simulink model "r_128w_8k_1a_16x_r431"  (R2012b)
settings: Solver=FixedStepDiscrete  SolverMode=SingleTasking  StartTime=0.0  StopTime=5000  RelTol=1e-3
undefined symbols (not defined in the file): Down, pfb_coeff_gen_calc, Up
libraries: xbsIndex_r4 x9410, casper_library_misc x257, casper_library_delays x92, xps_library x57, simulink x16, dspsigops x12, casper_library_flow_control x8, xbsReplacements_r4 x4, casper_library_multipliers x4, casper_library_scopes x2, casper_library_ffts_twiddle x2
(part 1 of 125)
settings Model: ExtModeAutoUpdateStatusClock=off  Creator=Jason Manley  LastModifiedBy=jmanley
settings DataIOCC: SignalLoggingSaveFormat=ModelDataLogs  SaveOutput=off  SaveTime=off
settings OptimizationCC: InitFltsAndDblsToZero=on
settings DebuggingCC: SolverPrmCheckMsg=none  FcnCallInpInsideContextMsg=UseLocalSettings  StrictBusMsg=Warning
settings GRTTargetCC: CombineOutputUpdateFcns=off  GRTInterface=on

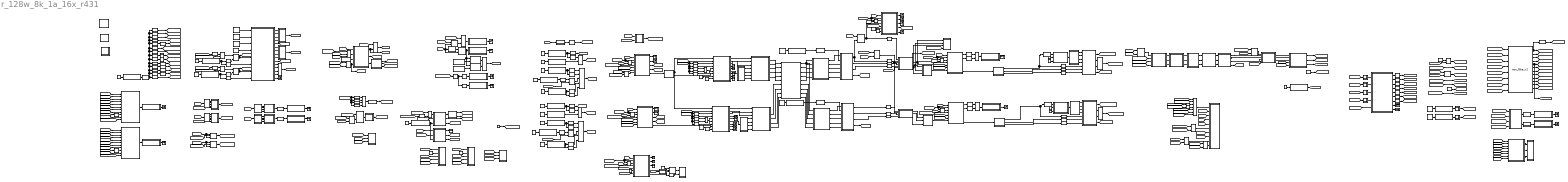
== system r_128w_8k_1a_16x_r431 ==
  note: * A resync command will cause the sync_gen to stop issuing sync pulses.
      | * It will then ignore the next input trigger (1PPS), while sync is flushed through the DSP pipeline.
      | * It will then lock onto the next trigger (1PPS) and issue a sync.
      | * Need a multiple of (pfb_fir taps*LCM(FFT reorder orders) *fft bins/parallel inputs =)
      | (4 * LCM(2,2,2,9) * 2048 / 4) = 9216) for sync_period for simulation
  note: coarse delay logic
  note: Prevent saturation
      | in first stage of FFT
      | by shifting down.
  note: Controls whether there is
      | a shift to the right after
      | multiplication at the
      | respective stage in the
      | fft to prevent
      | overflow.
  note: requantisation
      | to 4 bits
  note: polyphase FIR and FFT
  note: Accept 32 data words from ibob,
      | plus a 1 word header,
      | creating UDP packets of length 33 x 64 bits.
      | This block generates the destination IP address.
  note: Fine delay tracking and
      | fringe stopping
  note: delay tracking and
      | fringe stopping registers
  note: clock and synchronisation
      | info
  note: transient event/RFI debugging infrastructure
  note: data alignment infrastructure to
      | align to within one clock cycle
      | using PPS
  note: input power estimation
      | infrastructure
  note: ADC protection
      | infrastructure
  note: data reordering
  note: packet formation
  note: comms
  note: outputs value to GPIO pin to
      | prove timed register functionality
  note: tvg that can be activated at
      | specific time in data stream
  note: r431 2013-05-17
      | - 8k mode based on r430 1k mode
      | - 4taps
      | - new PFB
      | - new snap blocks
      | - new shared bram
      | - removed snap_xaui and snap_quant to save BRAM
  " System Generator" : xbsIndex_r4/ System Generator  Tag=genX  xilinxfamily=virtex5  part=xc5vsx95t  speed=-1  package=ff1136  synthesis_tool=XST  clock_wrapper=Clock Enables  directory=./r_128w_8k_1a_16x_r431/sysgen  proj_type=Project Navigator  Synth_file=XST Defaults  Impl_file=ISE Defaults  testbench=off  simulink_period=1  sysclk_period=5  dcm_input_clock_period=100  incr_netlist=off  trim_vbits=Everywhere in SubSystem  dbl_ovrd=According to Block Masks  core_generation=According to Block Masks  run_coregen=off  deprecated_control=off  eval_field=0  block_type=sysgen
      settings: block_version=10.1.3
  AddSub : xbsIndex_r4/AddSub  mode=Addition  use_carryin=off  use_carryout=off  en=off  latency=1  precision=User Defined  arith_type=Unsigned  n_bits=15  bin_pt=0  quantization=Truncate  overflow=Saturate  dbl_ovrd=off  use_behavioral_HDL=off  hw_selection=DSP48  pipelined=on  block_type=addsub
  AddSub1 : xbsIndex_r4/AddSub  mode=Addition  use_carryin=off  use_carryout=off  en=off  latency=1  precision=User Defined  arith_type=Unsigned  n_bits=15  bin_pt=0  quantization=Truncate  overflow=Saturate  dbl_ovrd=off  use_behavioral_HDL=off  hw_selection=DSP48  pipelined=on  block_type=addsub
  Concat : xbsIndex_r4/Concat  num_inputs=3  dbl_ovrd=off  block_type=concat
      settings: block_version=10.1.3
  Concat1 : xbsIndex_r4/Concat  num_inputs=5  dbl_ovrd=off  block_type=concat
      settings: block_version=10.1.3
  Concat{2..7,9..10,13..14,21} (11 alike) : xbsIndex_r4/Concat  num_inputs=2  dbl_ovrd=off  block_type=concat
      Concat13 settings: block_version=10.1.3
      Concat14 settings: block_version=10.1.3
      Concat2 settings: block_version=10.1.3
      Concat3 settings: block_version=10.1.3
      Concat7 settings: block_version=10.1.3
      Concat9 settings: block_version=10.1.3
  Concat22 : xbsIndex_r4/Concat  num_inputs=5  dbl_ovrd=off  block_type=concat
      settings: block_version=10.1.3
  Concat8 : xbsIndex_r4/Concat  num_inputs=4  dbl_ovrd=off  block_type=concat
  Constant : Constant  SampleTime=1/4
  Constant1 : xbsIndex_r4/Constant  const=1  gui_display_data_type=Fixed-point  arith_type=Boolean  n_bits=1  bin_pt=0  preci_type=Single  exp_width=8  frac_width=24  explicit_period=off  period=1  equ=P=C  opselect=C  inp2=PCIN>>17  opr=+  inp1=P  carry=CIN  dbl_ovrd=off  block_type=constant
      settings: block_version=11.4
  Constant10 : xbsIndex_r4/Constant  const=0  gui_display_data_type=Fixed-point  arith_type=Unsigned  n_bits=64  bin_pt=0  preci_type=Single  exp_width=8  frac_width=24  explicit_period=off  period=1  equ=P=C  opselect=C  inp2=PCIN>>17  opr=+  inp1=P  carry=CIN  dbl_ovrd=off  block_type=constant
      settings: block_version=11.4
  Constant11 : xbsIndex_r4/Constant  const=0  gui_display_data_type=Fixed-point  arith_type=Boolean  n_bits=64  bin_pt=0  preci_type=Single  exp_width=8  frac_width=24  explicit_period=off  period=1  equ=P=C  opselect=C  inp2=PCIN>>17  opr=+  inp1=P  carry=CIN  dbl_ovrd=off  block_type=constant
      settings: block_version=11.4
  Constant{4,8,12,15..16,32} (6 alike) : Constant  Value=8
  Constant{3,9,13,18,27,33,40,48} (8 alike) : Constant  Value=0
  Constant{14,19..20,22,35} (5 alike) : xbsIndex_r4/Constant  const=0  gui_display_data_type=Fixed-point  arith_type=Boolean  n_bits=1  bin_pt=0  preci_type=Single  exp_width=8  frac_width=24  explicit_period=on  period=1  equ=P=C  opselect=C  inp2=PCIN>>17  opr=+  inp1=P  carry=CIN  dbl_ovrd=off  block_type=constant
      Constant14 settings: block_version=11.4
      Constant19 settings: block_version=11.4
      Constant20 settings: block_version=11.3
      Constant22 settings: block_version=11.4
      Constant35 settings: block_version=11.4
  Constant17 : xbsIndex_r4/Constant  const=0  gui_display_data_type=Fixed-point  arith_type=Unsigned  n_bits=1  bin_pt=0  preci_type=Single  exp_width=8  frac_width=24  explicit_period=on  period=1  equ=P=C  opselect=C  inp2=PCIN>>17  opr=+  inp1=P  carry=CIN  dbl_ovrd=off  block_type=constant
      settings: block_version=11.4
  Constant2 : xbsIndex_r4/Constant  const=12*2*8192*2^14  gui_display_data_type=Fixed-point  arith_type=Unsigned  n_bits=32  bin_pt=0  preci_type=Single  exp_width=8  frac_width=24  explicit_period=off  period=1  equ=P=C  opselect=C  inp2=PCIN>>17  opr=+  inp1=P  carry=CIN  dbl_ovrd=off  block_type=constant
  Constant21 : xbsIndex_r4/Constant  const=0  gui_display_data_type=Fixed-point  arith_type=Unsigned  n_bits=1  bin_pt=0  preci_type=Single  exp_width=8  frac_width=24  explicit_period=on  period=1  equ=P=C  opselect=C  inp2=PCIN>>17  opr=+  inp1=P  carry=CIN  dbl_ovrd=off  block_type=constant
      settings: block_version=11.4
  Constant23 : xbsIndex_r4/Constant  const=0  gui_display_data_type=Boolean  arith_type=Boolean  n_bits=1  bin_pt=0  preci_type=Single  exp_width=8  frac_width=24  explicit_period=off  period=1  equ=P=C  opselect=C  inp2=PCIN>>17  opr=+  inp1=P  carry=CIN  dbl_ovrd=off  block_type=constant
      settings: block_version=11.4
  Constant24 : xbsIndex_r4/Constant  const=1  gui_display_data_type=Fixed-point  arith_type=Boolean  n_bits=1  bin_pt=0  preci_type=Single  exp_width=8  frac_width=24  explicit_period=off  period=1  equ=P=C  opselect=C  inp2=PCIN>>17  opr=+  inp1=P  carry=CIN  dbl_ovrd=off  block_type=constant
      settings: block_version=11.4
  Constant25 : Constant  Value=100
  Constant29 : Constant  Value=20
  Constant34 : xbsIndex_r4/Constant  const=0  gui_display_data_type=Fixed-point  arith_type=Boolean  n_bits=16  bin_pt=14  preci_type=Single  exp_width=8  frac_width=24  explicit_period=on  period=1  equ=P=C  opselect=C  inp2=PCIN>>17  opr=+  inp1=P  carry=CIN  dbl_ovrd=off  block_type=constant
      settings: block_version=11.4
  Constant36 : xbsIndex_r4/Constant  const=800000000/4+1  gui_display_data_type=Fixed-point  arith_type=Unsigned  n_bits=32  bin_pt=0  preci_type=Single  exp_width=8  frac_width=24  explicit_period=on  period=1  equ=P=C  opselect=C  inp2=PCIN>>17  opr=+  inp1=P  carry=CIN  dbl_ovrd=off  block_type=constant
      settings: block_version=11.4
  Constant37 : xbsIndex_r4/Constant  const=800000000/4-1  gui_display_data_type=Fixed-point  arith_type=Unsigned  n_bits=32  bin_pt=0  preci_type=Single  exp_width=8  frac_width=24  explicit_period=on  period=1  equ=P=C  opselect=C  inp2=PCIN>>17  opr=+  inp1=P  carry=CIN  dbl_ovrd=off  block_type=constant
      settings: block_version=11.4
  Constant38 : xbsIndex_r4/Constant  const=1  gui_display_data_type=Fixed-point  arith_type=Unsigned  n_bits=1  bin_pt=0  preci_type=Single  exp_width=8  frac_width=24  explicit_period=on  period=1  equ=P=C  opselect=C  inp2=PCIN>>17  opr=+  inp1=P  carry=CIN  dbl_ovrd=off  block_type=constant
      settings: block_version=11.4
  Constant41 : xbsIndex_r4/Constant  const=0  gui_display_data_type=Fixed-point  arith_type=Unsigned  n_bits=64  bin_pt=0  preci_type=Single  exp_width=8  frac_width=24  explicit_period=off  period=1  equ=P=C  opselect=C  inp2=PCIN>>17  opr=+  inp1=P  carry=CIN  dbl_ovrd=off  block_type=constant
      settings: block_version=11.4
  Constant46 : xbsIndex_r4/Constant  const=0  gui_display_data_type=Fixed-point  arith_type=Boolean  n_bits=64  bin_pt=0  preci_type=Single  exp_width=8  frac_width=24  explicit_period=off  period=1  equ=P=C  opselect=C  inp2=PCIN>>17  opr=+  inp1=P  carry=CIN  dbl_ovrd=off  block_type=constant
      settings: block_version=11.4
  Constant5 : xbsIndex_r4/Constant  const=1  gui_display_data_type=Fixed-point  arith_type=Boolean  n_bits=1  bin_pt=0  preci_type=Single  exp_width=8  frac_width=24  explicit_period=on  period=1  equ=P=C  opselect=C  inp2=PCIN>>17  opr=+  inp1=P  carry=CIN  dbl_ovrd=off  block_type=constant
  Constant6 : Constant  Value=20
  Constant7 : xbsIndex_r4/Constant  const=0  gui_display_data_type=Fixed-point  arith_type=Boolean  n_bits=16  bin_pt=14  preci_type=Single  exp_width=8  frac_width=24  explicit_period=on  period=1  equ=P=C  opselect=C  inp2=PCIN>>17  opr=+  inp1=P  carry=CIN  dbl_ovrd=off  block_type=constant
      settings: block_version=11.4
  Convert{4..7} (4 alike) : xbsIndex_r4/Convert  gui_display_data_type=Fixed-point  arith_type=Unsigned  n_bits=16  bin_pt=0  float_type=Single  exp_bits=8  fraction_bits=24  quantization=Truncate  overflow=Wrap  en=off  latency=0  dbl_ovrd=off  pipeline=on  block_type=convert
      settings: block_version=11.4
  Counter1 : xbsIndex_r4/Counter  cnt_type=Free Running  cnt_to=Inf  operation=Up  start_count=1  cnt_by_val=1  arith_type=Unsigned  n_bits=32  bin_pt=0  load_pin=off  rst=on  en=off  explicit_period=on  period=1  dbl_ovrd=off  use_behavioral_HDL=off  implementation=Fabric  use_rpm=on  block_type=counter
  Counter2 : xbsIndex_r4/Counter  cnt_type=Free Running  cnt_to=Inf  operation=Up  start_count=0  cnt_by_val=1  arith_type=Unsigned  n_bits=12  bin_pt=0  load_pin=off  rst=on  en=off  explicit_period=on  period=1  dbl_ovrd=off  use_behavioral_HDL=off  implementation=Fabric  block_type=counter
      settings: block_version=11.4
  Counter3 : xbsIndex_r4/Counter  cnt_type=Free Running  cnt_to=Inf  operation=Up  start_count=0  cnt_by_val=1  arith_type=Unsigned  n_bits=31  bin_pt=0  load_pin=off  rst=on  en=on  explicit_period=on  period=1  dbl_ovrd=off  use_behavioral_HDL=off  implementation=DSP48  use_rpm=on  block_type=counter
  Counter8 : xbsIndex_r4/Counter  cnt_type=Free Running  cnt_to=Inf  operation=Up  start_count=0  cnt_by_val=1  arith_type=Unsigned  n_bits=12  bin_pt=0  load_pin=off  rst=on  en=off  explicit_period=on  period=1  dbl_ovrd=off  use_behavioral_HDL=off  implementation=Fabric  block_type=counter
      settings: block_version=11.4
  Delay : xbsIndex_r4/Delay  rst=off  infoeditControl=Selection of Reset will increase slice count due to use of real FFs and instead of SRLs  en=off  latency=1  dbl_ovrd=off  reg_retiming=off  block_type=delay
      settings: block_version=11.4
  Delay1 : Subsystem  AncestorBlock=casper_library/Delays/pipeline  mask(pipeline){latency=1}
      mask help:
      | An explicitly laid-out delay line to avoid mapping to SRL16s
      | for use in pipelining to help achieve timing closure.
      mask init:
      | pipeline_init(gcb, 'latency', latency);
      mask Display:
      | port_label('input', 1, 'd');
      | port_label('output', 1, 'q');
      | disp(['Z^-', num2str(latency)]);
  Delay10 : Subsystem  AncestorBlock=casper_library/Delays/pipeline  mask(pipeline){latency=1}
      mask help:
      | An explicitly laid-out delay line to avoid mapping to SRL16s
      | for use in pipelining to help achieve timing closure.
      mask init:
      | pipeline_init(gcb, 'latency', latency);
      mask Display:
      | port_label('input', 1, 'd');
      | port_label('output', 1, 'q');
      | disp(['Z^-', num2str(latency)]);
  Delay100 : Subsystem  AncestorBlock=casper_library/Delays/pipeline  mask(pipeline){latency=2}
      mask help:
      | An explicitly laid-out delay line to avoid mapping to SRL16s
      | for use in pipelining to help achieve timing closure.
      mask init:
      | pipeline_init(gcb, 'latency', latency);
      mask Display:
      | port_label('input', 1, 'd');
      | port_label('output', 1, 'q');
      | disp(['Z^-', num2str(latency)]);
  Delay11 : Subsystem  AncestorBlock=casper_library/Delays/pipeline  mask(pipeline){latency=1}
      mask help:
      | An explicitly laid-out delay line to avoid mapping to SRL16s
      | for use in pipelining to help achieve timing closure.
      mask init:
      | pipeline_init(gcb, 'latency', latency);
      mask Display:
      | port_label('input', 1, 'd');
      | port_label('output', 1, 'q');
      | disp(['Z^-', num2str(latency)]);
  Delay12 : xbsIndex_r4/Delay  rst=off  infoeditControl=Selection of Reset will increase slice count due to use of real FFs and instead of SRLs  en=off  latency=1  dbl_ovrd=off  reg_retiming=off  block_type=delay
      settings: block_version=11.4
  Delay{13,15..19} (6 alike) : xbsIndex_r4/Delay  rst=off  infoeditControl=Selection of Reset will increase slice count due to use of real FFs and instead of SRLs  en=off  latency=3  dbl_ovrd=off  reg_retiming=off  block_type=delay
      settings: block_version=11.4
  Delay14 : Subsystem  AncestorBlock=casper_library/Delays/pipeline  mask(pipeline){latency=2}
      mask help:
      | An explicitly laid-out delay line to avoid mapping to SRL16s
      | for use in pipelining to help achieve timing closure.
      mask init:
      | pipeline_init(gcb, 'latency', latency);
      mask Display:
      | port_label('input', 1, 'd');
      | port_label('output', 1, 'q');
      | disp(['Z^-', num2str(latency)]);
  Delay2 : Subsystem  AncestorBlock=casper_library/Delays/pipeline  mask(pipeline){latency=2}
      mask help:
      | An explicitly laid-out delay line to avoid mapping to SRL16s
      | for use in pipelining to help achieve timing closure.
      mask init:
      | pipeline_init(gcb, 'latency', latency);
      mask Display:
      | port_label('input', 1, 'd');
      | port_label('output', 1, 'q');
      | disp(['Z^-', num2str(latency)]);
  Delay{20..22,24..27} (7 alike) : xbsIndex_r4/Delay  rst=off  infoeditControl=Selection of Reset will increase slice count due to use of real FFs and instead of SRLs  en=off  latency=4  dbl_ovrd=off  reg_retiming=off  block_type=delay
      settings: block_version=11.4
  Delay23 : Subsystem  AncestorBlock=casper_library/Delays/pipeline  mask(pipeline){latency=1}
      mask help:
      | An explicitly laid-out delay line to avoid mapping to SRL16s
      | for use in pipelining to help achieve timing closure.
      mask init:
      | pipeline_init(gcb, 'latency', latency);
      mask Display:
      | port_label('input', 1, 'd');
      | port_label('output', 1, 'q');
      | disp(['Z^-', num2str(latency)]);
  Delay28 : xbsIndex_r4/Delay  rst=off  infoeditControl=Selection of Reset will increase slice count due to use of real FFs and instead of SRLs  en=off  latency=1  dbl_ovrd=off  reg_retiming=on  block_type=delay
  Delay3 : Subsystem  AncestorBlock=casper_library/Delays/pipeline  mask(pipeline){latency=1}
      mask help:
      | An explicitly laid-out delay line to avoid mapping to SRL16s
      | for use in pipelining to help achieve timing closure.
      mask init:
      | pipeline_init(gcb, 'latency', latency);
      mask Display:
      | port_label('input', 1, 'd');
      | port_label('output', 1, 'q');
      | disp(['Z^-', num2str(latency)]);
  Delay31 : Subsystem  AncestorBlock=casper_library/Delays/pipeline  mask(pipeline){latency=1}
      mask help:
      | An explicitly laid-out delay line to avoid mapping to SRL16s
      | for use in pipelining to help achieve timing closure.
      mask init:
      | pipeline_init(gcb, 'latency', latency);
      mask Display:
      | port_label('input', 1, 'd');
      | port_label('output', 1, 'q');
      | disp(['Z^-', num2str(latency)]);
  Delay33 : Subsystem  AncestorBlock=casper_library/Delays/pipeline  mask(pipeline){latency=1}
      mask help:
      | An explicitly laid-out delay line to avoid mapping to SRL16s
      | for use in pipelining to help achieve timing closure.
      mask init:
      | pipeline_init(gcb, 'latency', latency);
      mask Display:
      | port_label('input', 1, 'd');
      | port_label('output', 1, 'q');
      | disp(['Z^-', num2str(latency)]);
  Delay34 : Subsystem  AncestorBlock=casper_library/Delays/pipeline  mask(pipeline){latency=1}
      mask help:
      | An explicitly laid-out delay line to avoid mapping to SRL16s
      | for use in pipelining to help achieve timing closure.
      mask init:
      | pipeline_init(gcb, 'latency', latency);
      mask Display:
      | port_label('input', 1, 'd');
      | port_label('output', 1, 'q');
      | disp(['Z^-', num2str(latency)]);
  Delay4 : Subsystem  AncestorBlock=casper_library/Delays/pipeline  mask(pipeline){latency=1}
      mask help:
      | An explicitly laid-out delay line to avoid mapping to SRL16s
      | for use in pipelining to help achieve timing closure.
      mask init:
      | pipeline_init(gcb, 'latency', latency);
      mask Display:
      | port_label('input', 1, 'd');
      | port_label('output', 1, 'q');
      | disp(['Z^-', num2str(latency)]);
  Delay5 : Subsystem  AncestorBlock=casper_library/Delays/pipeline  mask(pipeline){latency=1}
      mask help:
      | An explicitly laid-out delay line to avoid mapping to SRL16s
      | for use in pipelining to help achieve timing closure.
      mask init:
      | pipeline_init(gcb, 'latency', latency);
      mask Display:
      | port_label('input', 1, 'd');
      | port_label('output', 1, 'q');
      | disp(['Z^-', num2str(latency)]);
  Delay6 : xbsIndex_r4/Delay  rst=off  infoeditControl=Selection of Reset will increase slice count due to use of real FFs and instead of SRLs  en=off  latency=1  dbl_ovrd=off  reg_retiming=on  block_type=delay
  Delay64 : Subsystem  AncestorBlock=casper_library/Delays/pipeline  mask(pipeline){latency=2}
      mask help:
      | An explicitly laid-out delay line to avoid mapping to SRL16s
      | for use in pipelining to help achieve timing closure.
      mask init:
      | pipeline_init(gcb, 'latency', latency);
      mask Display:
      | port_label('input', 1, 'd');
      | port_label('output', 1, 'q');
      | disp(['Z^-', num2str(latency)]);
  Delay7 : xbsIndex_r4/Delay  rst=off  infoeditControl=Selection of Reset will increase slice count due to use of real FFs and instead of SRLs  en=off  latency=1  dbl_ovrd=off  reg_retiming=on  block_type=delay
  Delay71 : Subsystem  AncestorBlock=casper_library/Delays/pipeline  mask(pipeline){latency=2}
      mask help:
      | An explicitly laid-out delay line to avoid mapping to SRL16s
      | for use in pipelining to help achieve timing closure.
      mask init:
      | pipeline_init(gcb, 'latency', latency);
      mask Display:
      | port_label('input', 1, 'd');
      | port_label('output', 1, 'q');
      | disp(['Z^-', num2str(latency)]);
  Delay72 : Subsystem  AncestorBlock=casper_library/Delays/pipeline  mask(pipeline){latency=2}
      mask help:
      | An explicitly laid-out delay line to avoid mapping to SRL16s
      | for use in pipelining to help achieve timing closure.
      mask init:
      | pipeline_init(gcb, 'latency', latency);
      mask Display:
      | port_label('input', 1, 'd');
      | port_label('output', 1, 'q');
      | disp(['Z^-', num2str(latency)]);
  Delay8 : xbsIndex_r4/Delay  rst=off  infoeditControl=Selection of Reset will increase slice count due to use of real FFs and instead of SRLs  en=off  latency=1  dbl_ovrd=off  reg_retiming=off  block_type=delay
      settings: block_version=11.4
  Delay9 : Subsystem  AncestorBlock=casper_library/Delays/pipeline  mask(pipeline){latency=1}
      mask help:
      | An explicitly laid-out delay line to avoid mapping to SRL16s
      | for use in pipelining to help achieve timing closure.
      mask init:
      | pipeline_init(gcb, 'latency', latency);
      mask Display:
      | port_label('input', 1, 'd');
      | port_label('output', 1, 'q');
      | disp(['Z^-', num2str(latency)]);
  Inverter{,1..6} (7 alike) : xbsIndex_r4/Inverter  en=off  latency=0  dbl_ovrd=off  block_type=inv
      settings: block_version=11.4
  Logical : xbsIndex_r4/Logical  logical_function=OR  inputs=4  en=off  latency=0  precision=Full  arith_type=Unsigned  n_bits=16  bin_pt=0  align_bp=on  dbl_ovrd=off  block_type=logical
  Logical1 : xbsIndex_r4/Logical  logical_function=AND  inputs=2  en=off  latency=0  precision=Full  arith_type=Unsigned  n_bits=8  bin_pt=2  align_bp=on  dbl_ovrd=off  block_type=logical
      settings: xl_area=[0, 0, 0, 0, 0, 0, 0]
  Logical10 : xbsIndex_r4/Logical  logical_function=AND  inputs=2  en=off  latency=0  precision=Full  arith_type=Unsigned  n_bits=16  bin_pt=0  align_bp=on  dbl_ovrd=off  block_type=logical
  Logical{3..4,6,9,11..15,19..21} (12 alike) : xbsIndex_r4/Logical  logical_function=OR  inputs=2  en=off  latency=0  precision=Full  arith_type=Unsigned  n_bits=16  bin_pt=0  align_bp=on  dbl_ovrd=off  block_type=logical
      Logical11 settings: block_version=11.4
      Logical12 settings: block_version=11.4
      Logical13 settings: block_version=11.4
      Logical15 settings: block_version=11.4
      Logical19 settings: block_version=11.4
      Logical20 settings: block_version=11.4
      Logical21 settings: block_version=11.4
  Logical16 : xbsIndex_r4/Logical  logical_function=OR  inputs=2  en=off  latency=1  precision=Full  arith_type=Unsigned  n_bits=16  bin_pt=0  align_bp=on  dbl_ovrd=off  block_type=logical
  Logical17 : xbsIndex_r4/Logical  logical_function=OR  inputs=2  en=off  latency=1  precision=Full  arith_type=Unsigned  n_bits=16  bin_pt=0  align_bp=on  dbl_ovrd=off  block_type=logical
  Logical2 : xbsIndex_r4/Logical  logical_function=OR  inputs=2  en=off  latency=1  precision=Full  arith_type=Unsigned  n_bits=8  bin_pt=2  align_bp=on  dbl_ovrd=off  block_type=logical
      settings: xl_area=[0, 0, 0, 0, 0, 0, 0]
  Logical5 : xbsIndex_r4/Logical  logical_function=AND  inputs=2  en=off  latency=0  precision=Full  arith_type=Unsigned  n_bits=16  bin_pt=0  align_bp=on  dbl_ovrd=off  block_type=logical
  Logical7 : xbsIndex_r4/Logical  logical_function=OR  inputs=7  en=off  latency=1  precision=Full  arith_type=Unsigned  n_bits=16  bin_pt=0  align_bp=on  dbl_ovrd=off  block_type=logical
  Logical8 : xbsIndex_r4/Logical  logical_function=AND  inputs=2  en=off  latency=0  precision=Full  arith_type=Unsigned  n_bits=16  bin_pt=0  align_bp=on  dbl_ovrd=off  block_type=logical
  Pulse Generator : DiscretePulseGenerator  Amplitude=0.75  Period=2^11  PhaseDelay=11  SampleTime=1/4
  Pulse Generator1 : DiscretePulseGenerator  Period=2^8  PhaseDelay=9+13+2^8  SampleTime=1/4
  Pulse Generator2 : DiscretePulseGenerator  Amplitude=0.5  Period=2^11  PhaseDelay=9+14+2^8  SampleTime=1/4
  Recombine channels : Subsystem  mask{channel_bits=8}
      mask prompts: channel_bits "Bits per channel:"
      mask help: FFT data per polarisation is in the form of two channels of n-bit data concatenated together. This block splits given inputs of this form and groups outputs by channel, not polarisation.
  Register{,1..3,19} (5 alike) : xbsIndex_r4/Register  init=0  rst=off  en=on  dbl_ovrd=off  block_type=register
      Register settings: block_version=11.4
      Register1 settings: block_version=11.4
      Register2 settings: block_version=11.4
      Register3 settings: block_version=11.4
  Register4 : xbsIndex_r4/Register  init=0  rst=on  en=on  dbl_ovrd=off  block_type=register
      settings: block_version=11.4
  Register5 : xbsIndex_r4/Register  init=0  rst=on  en=on  dbl_ovrd=off  block_type=register
  Register9 : xbsIndex_r4/Register  init=0  rst=on  en=on  dbl_ovrd=off  block_type=register
  Relational : xbsIndex_r4/Relational  mode=a>b  en=off  latency=1  dbl_ovrd=off  block_type=relational
  Relational1 : xbsIndex_r4/Relational  mode=a<b  en=off  latency=1  dbl_ovrd=off  block_type=relational
  Slice : xbsIndex_r4/Slice  nbits=32  boolean_output=off  mode=Lower Bit Location + Width  bit1=0  base1=MSB of Input  bit0=0  base0=LSB of Input  dbl_ovrd=off  block_type=slice
  Slice1 : xbsIndex_r4/Slice  nbits=32  boolean_output=off  mode=Lower Bit Location + Width  bit1=0  base1=MSB of Input  bit0=32  base0=LSB of Input  dbl_ovrd=off  block_type=slice
  Slice{2,4,13,28,37,73} (6 alike) : xbsIndex_r4/Slice  nbits=16  boolean_output=off  mode=Lower Bit Location + Width  bit1=0  base1=MSB of Input  bit0=0  base0=LSB of Input  dbl_ovrd=off  block_type=slice
      settings: infoedit="Extracts a given range of bits from each input sample and presents it at the output.  The output type is ordinarily unsigned with binary point at zero, but can be Boolean when the slice is one bit wide.<P><P>Hardware notes: In hardware this block costs nothing."  block_version=10.1.3
  Slice14 : xbsIndex_r4/Slice  nbits=32  boolean_output=off  mode=Lower Bit Location + Width  bit1=0  base1=MSB of Input  bit0=0  base0=LSB of Input  dbl_ovrd=off  block_type=slice
  Slice15 : xbsIndex_r4/Slice  nbits=16  boolean_output=off  mode=Lower Bit Location + Width  bit1=0  base1=MSB of Input  bit0=0*16  base0=LSB of Input  dbl_ovrd=off  block_type=slice
      settings: block_version=10.1.3
  Slice16 : xbsIndex_r4/Slice  nbits=16  boolean_output=off  mode=Lower Bit Location + Width  bit1=0  base1=MSB of Input  bit0=16*3+15  base0=LSB of Input  dbl_ovrd=off  block_type=slice
      settings: block_version=10.1.3
  Slice17 : xbsIndex_r4/Slice  nbits=16  boolean_output=off  mode=Lower Bit Location + Width  bit1=0  base1=MSB of Input  bit0=16*1  base0=LSB of Input  dbl_ovrd=off  block_type=slice
      settings: block_version=10.1.3
  Slice18 : xbsIndex_r4/Slice  nbits=15  boolean_output=off  mode=Lower Bit Location + Width  bit1=0  base1=MSB of Input  bit0=16*2  base0=LSB of Input  dbl_ovrd=off  block_type=slice
      settings: block_version=10.1.3
  Slice19 : xbsIndex_r4/Slice  nbits=16  boolean_output=off  mode=Lower Bit Location + Width  bit1=0  base1=MSB of Input  bit0=16*2+15  base0=LSB of Input  dbl_ovrd=off  block_type=slice
      settings: block_version=10.1.3
  Slice20 : xbsIndex_r4/Slice  nbits=16  boolean_output=off  mode=Lower Bit Location + Width  bit1=0  base1=MSB of Input  bit0=0*16  base0=LSB of Input  dbl_ovrd=off  block_type=slice
      settings: block_version=10.1.3
  Slice21 : xbsIndex_r4/Slice  nbits=16  boolean_output=off  mode=Lower Bit Location + Width  bit1=0  base1=MSB of Input  bit0=16*3+15  base0=LSB of Input  dbl_ovrd=off  block_type=slice
      settings: block_version=10.1.3
  Slice22 : xbsIndex_r4/Slice  nbits=16  boolean_output=off  mode=Lower Bit Location + Width  bit1=0  base1=MSB of Input  bit0=16*1  base0=LSB of Input  dbl_ovrd=off  block_type=slice
      settings: block_version=10.1.3
  Slice23 : xbsIndex_r4/Slice  nbits=15  boolean_output=off  mode=Lower Bit Location + Width  bit1=0  base1=MSB of Input  bit0=16*2  base0=LSB of Input  dbl_ovrd=off  block_type=slice
      settings: block_version=10.1.3
  Slice24 : xbsIndex_r4/Slice  nbits=16  boolean_output=off  mode=Lower Bit Location + Width  bit1=0  base1=MSB of Input  bit0=16*2+15  base0=LSB of Input  dbl_ovrd=off  block_type=slice
      settings: block_version=10.1.3
  Slice{3,5,25,31} (4 alike) : xbsIndex_r4/Slice  nbits=16  boolean_output=off  mode=Lower Bit Location + Width  bit1=0  base1=MSB of Input  bit0=16  base0=LSB of Input  dbl_ovrd=off  block_type=slice
      Slice25 settings: infoedit="Extracts a given range of bits from each input sample and presents it at the output.  The output type is ordinarily unsigned with binary point at zero, but can be Boolean when the slice is one bit wide.<P><P>Hardware notes: In hardware this block costs nothing."  block_version=10.1.3
      Slice3 settings: infoedit="Extracts a given range of bits from each input sample and presents it at the output.  The output type is ordinarily unsigned with binary point at zero, but can be Boolean when the slice is one bit wide.<P><P>Hardware notes: In hardware this block costs nothing."  block_version=10.1.3
      Slice31 settings: block_version=10.1.3
      Slice5 settings: block_version=10.1.3
  Slice{6,26..27,38} (4 alike) : xbsIndex_r4/Slice  nbits=15  boolean_output=off  mode=Lower Bit Location + Width  bit1=0  base1=MSB of Input  bit0=0  base0=LSB of Input  dbl_ovrd=off  block_type=slice
      settings: block_version=10.1.3
  Slice{7,29,32..33} (4 alike) : xbsIndex_r4/Slice  nbits=1  boolean_output=on  mode=Upper Bit Location + Width  bit1=0  base1=MSB of Input  bit0=0  base0=LSB of Input  dbl_ovrd=off  block_type=slice
      Slice32 settings: block_version=10.1.3
      Slice7 settings: block_version=10.1.3
  Slice30 : xbsIndex_r4/Slice  nbits=6  boolean_output=off  mode=Lower Bit Location + Width  bit1=0  base1=MSB of Input  bit0=0  base0=LSB of Input  dbl_ovrd=off  block_type=slice
  Slice34 : xbsIndex_r4/Slice  nbits=6  boolean_output=off  mode=Lower Bit Location + Width  bit1=0  base1=MSB of Input  bit0=0  base0=LSB of Input  dbl_ovrd=off  block_type=slice
  Slice35 : xbsIndex_r4/Slice  nbits=1  boolean_output=on  mode=Lower Bit Location + Width  bit1=0  base1=MSB of Input  bit0=3  base0=LSB of Input  dbl_ovrd=off  block_type=slice
  Slice36 : xbsIndex_r4/Slice  nbits=1  boolean_output=on  mode=Lower Bit Location + Width  bit1=0  base1=MSB of Input  bit0=2  base0=LSB of Input  dbl_ovrd=off  block_type=slice
  Slice40 : xbsIndex_r4/Slice  nbits=1  boolean_output=on  mode=Lower Bit Location + Width  bit1=0  base1=MSB of Input  bit0=1  base0=LSB of Input  dbl_ovrd=off  block_type=slice
  Slice45 : xbsIndex_r4/Slice  nbits=1  boolean_output=on  mode=Lower Bit Location + Width  bit1=0  base1=MSB of Input  bit0=0  base0=LSB of Input  dbl_ovrd=off  block_type=slice
  Slice78 : xbsIndex_r4/Slice  nbits=1  boolean_output=on  mode=Lower Bit Location + Width  bit1=0  base1=MSB of Input  bit0=0  base0=LSB of Input  dbl_ovrd=off  block_type=slice
      settings: block_version=10.1.3
  Split channels : Subsystem  mask{channel_bits=8}
      mask prompts: channel_bits "Bits per channel:"
      mask help: FFT data per polarisation is in the form of two channels of n-bit data concatenated together. This block splits given inputs of this form and groups outputs by channel, not polarisation.
  Subsystem1 : Subsystem
  Subsystem3 : Subsystem
  Subsystem4 : Subsystem
  Subsystem5 : Subsystem
  Subsystem7 : Subsystem
  Terminator{,1..19,21,23,25..29,35..44} (37 alike) : Terminator
  X-engine reorder : Subsystem  mask{num_channels_bits=13, num_xengines_bits=4, num_data_bits=16, bram_latency=0}
      mask prompts: num_channels_bits "Number of channels (2^?)"; num_xengines_bits "Number of X-engines (2^?)"; num_data_bits "Incoming data width in bits (per channel, 2 pols):"; bram_latency "BRAM latency"
      mask help:
      | Interleaves the parallel output (even and odd channels) of an FFT between multiple X-engines in a correlator.
      | i.e. X0 will get F0, F1, F2... and Xn will get F(nChan/nXeng), F(nChan/nXeng) + 1, etc.
  XSG core config : xps_library/XSG core config  Tag=xps:xsg  hw_sys=ROACH:sx95t  clk_src=adc0_clk  ROACH_clk_src=adc0_clk  ROACH2_clk_src=adc0_clk  clk_rate=800/4  sample_period=1  synthesis_tool=XST
  a0_fd0 : xps_library/software register  Tag=xps:sw_reg  io_dir=From Processor  arith_type=Unsigned  bitwidth=32  bin_pt=0  sample_period=1  gw_name=r_128w_8k_1a_16x_r431_a0_fd0_user_data_out
      link override r_128w_8k_1a_16x_r430_a0_fd0_user_data_out: arith_type=Unsigned  n_bits=32  bin_pt=0  period=1
      link override r_128w_8k_1a_16x_r431_a0_fd0_user_data_out: arith_type=Unsigned  n_bits=32  bin_pt=0  period=1
  a0_fd1 : xps_library/software register  Tag=xps:sw_reg  io_dir=From Processor  arith_type=Unsigned  bitwidth=32  bin_pt=0  sample_period=1  gw_name=r_128w_8k_1a_16x_r431_a0_fd1_user_data_out
      link override r_128w_8k_1a_16x_r430_a0_fd1_user_data_out: arith_type=Unsigned  n_bits=32  bin_pt=0  period=1
      link override r_128w_8k_1a_16x_r431_a0_fd1_user_data_out: arith_type=Unsigned  n_bits=32  bin_pt=0  period=1
  a0p0_1st_shift : Subsystem  mask{shift=1, latency=0}
      mask prompts: shift "Number bits to shift right by"; latency "Shift latency"
  a0p1_1st_shift : Subsystem  mask{shift=1, latency=0}
      mask prompts: shift "Number bits to shift right by"; latency "Shift latency"
  a1_fd0 : xps_library/software register  Tag=xps:sw_reg  io_dir=From Processor  arith_type=Unsigned  bitwidth=32  bin_pt=0  sample_period=1  gw_name=r_128w_8k_1a_16x_r431_a1_fd0_user_data_out
      link override r_128w_8k_1a_16x_r430_a1_fd0_user_data_out: arith_type=Unsigned  n_bits=32  bin_pt=0  period=1
      link override r_128w_8k_1a_16x_r431_a1_fd0_user_data_out: arith_type=Unsigned  n_bits=32  bin_pt=0  period=1
  a1_fd1 : xps_library/software register  Tag=xps:sw_reg  io_dir=From Processor  arith_type=Unsigned  bitwidth=32  bin_pt=0  sample_period=1  gw_name=r_128w_8k_1a_16x_r431_a1_fd1_user_data_out
      link override r_128w_8k_1a_16x_r430_a1_fd1_user_data_out: arith_type=Unsigned  n_bits=32  bin_pt=0  period=1
      link override r_128w_8k_1a_16x_r431_a1_fd1_user_data_out: arith_type=Unsigned  n_bits=32  bin_pt=0  period=1
  adc_ctrl0 : xps_library/software register  Tag=xps:sw_reg  io_dir=From Processor  arith_type=Unsigned  bitwidth=32  bin_pt=0  sample_period=1  gw_name=r_128w_8k_1a_16x_r431_adc_ctrl0_user_data_out
      link override r_128w_8k_1a_16x_r430_adc_ctrl0_user_data_out: arith_type=Unsigned  n_bits=32  bin_pt=0  period=1
      link override r_128w_8k_1a_16x_r431_adc_ctrl0_user_data_out: arith_type=Unsigned  n_bits=32  bin_pt=0  period=1
  adc_ctrl1 : xps_library/software register  Tag=xps:sw_reg  io_dir=From Processor  arith_type=Unsigned  bitwidth=32  bin_pt=0  sample_period=1  gw_name=r_128w_8k_1a_16x_r431_adc_ctrl1_user_data_out
      link override r_128w_8k_1a_16x_r430_adc_ctrl1_user_data_out: arith_type=Unsigned  n_bits=32  bin_pt=0  period=1
      link override r_128w_8k_1a_16x_r431_adc_ctrl1_user_data_out: arith_type=Unsigned  n_bits=32  bin_pt=0  period=1
  adc_scope : Subsystem
  adc_snap0 : Subsystem  Tag=casper:snapshot  AncestorBlock=casper_library_scopes/snapshot  mask(snapshot){storage=bram, dram_dimm=1, dram_clock=200, nsamples=11, data_width=32, offset=on, circap=on, value=on, use_dsp48=off}
      mask prompts: storage "Storage medium"; dram_dimm "DRAM dimm"; dram_clock "DRAM clock rate"; nsamples "Number of Samples (2^?)"; data_width "Data width"; offset "Start delay support"; circap "Circular capture support"; value "Extra value capture support"; use_dsp48 "Use DSP48s to implement counters"
      mask help:
      | Standard snap block, but with the following optional extras;
      |  1) Optionally delay the fabric trigger by a user-specified number of valids.
      |  2) Capture continuously after a trigger until a stop pulse is received. Data is captured into BRAM continuously, with old data being overwritten until a stop command is received. Then stop capturing when memory is filled. This enables you to get some data before and some data after the stop pulse. Use the 'tr_en_cnt' register to determine where you are in your vector. 'Addr' register's MSb now indicates 'busy capturing'.
      |  3) Optionally capture a value on an input port to a register at the same time as the first data sample.
      |  4) Implement counters using DSP48Es to save resources.
      mask init:
      | snapshot_init(gcb, ...
      |     'storage', storage, ...
      |     'dram_dimm', dram_dimm, ...
      |     'dram_clock', dram_clock, ...
      |     'nsamples', nsamples, ...
      |     'data_width', data_width, ...
      |     'offset', offset, ...
      |     'circap', circap, ...
      |     'value', value, ...
      |     'use_dsp48', use_dsp48);
      mask TypeOptions storage: bram | dram
      mask Callback storage: snapshot_callback();
      mask TypeOptions dram_dimm: 1 | 2 | 3 | 4
      mask TypeOptions dram_clock: 200 | 250 | 266 | 300 | 333
      mask TypeOptions data_width: 8 | 16 | 32 | 64 | 128
  adc_snap1 : Subsystem  Tag=casper:snapshot  AncestorBlock=casper_library_scopes/snapshot  mask(snapshot){storage=bram, dram_dimm=1, dram_clock=200, nsamples=11, data_width=32, offset=on, circap=on, value=on, use_dsp48=off}
      mask prompts: storage "Storage medium"; dram_dimm "DRAM dimm"; dram_clock "DRAM clock rate"; nsamples "Number of Samples (2^?)"; data_width "Data width"; offset "Start delay support"; circap "Circular capture support"; value "Extra value capture support"; use_dsp48 "Use DSP48s to implement counters"
      mask help:
      | Standard snap block, but with the following optional extras;
      |  1) Optionally delay the fabric trigger by a user-specified number of valids.
      |  2) Capture continuously after a trigger until a stop pulse is received. Data is captured into BRAM continuously, with old data being overwritten until a stop command is received. Then stop capturing when memory is filled. This enables you to get some data before and some data after the stop pulse. Use the 'tr_en_cnt' register to determine where you are in your vector. 'Addr' register's MSb now indicates 'busy capturing'.
      |  3) Optionally capture a value on an input port to a register at the same time as the first data sample.
      |  4) Implement counters using DSP48Es to save resources.
      mask init: same as r_128w_8k_1a_16x_r431/adc_snap0
      mask TypeOptions storage: bram | dram
      mask Callback storage: snapshot_callback();
      mask TypeOptions dram_dimm: 1 | 2 | 3 | 4
      mask TypeOptions dram_clock: 200 | 250 | 266 | 300 | 333
      mask TypeOptions data_width: 8 | 16 | 32 | 64 | 128
  adc_sum_sq0 : Subsystem  Tag=xps:sw_reg  mask{io_dir=To Processor, arith_type=Unsigned, bitwidth=32, bin_pt=0, sample_period=1, latency=0}
      mask prompts: io_dir "I/O direction"; arith_type "Data Type"; bitwidth "Data bitwidth"; bin_pt "Data binary point"; sample_period "Sample period"
      mask init:
      | gw_name = clear_name(gcb);
      | config.source = str2func('software_register_init');
      | config.toplevel = gcb;
      | xBlock( config, {io_dir, arith_type, bitwidth, bin_pt, ... 
      |     sample_period, gw_name, latency});
      mask TypeOptions io_dir: From Processor | To Processor
      mask TypeOptions arith_type: Unsigned | Signed  (2's comp)
  adc_sum_sq1 : Subsystem  Tag=xps:sw_reg  mask{io_dir=To Processor, arith_type=Unsigned, bitwidth=32, bin_pt=0, sample_period=1, latency=0}
      mask prompts: io_dir "I/O direction"; arith_type "Data Type"; bitwidth "Data bitwidth"; bin_pt "Data binary point"; sample_period "Sample period"
      mask init:
      | gw_name = clear_name(gcb);
      | config.source = str2func('software_register_init');
      | config.toplevel = gcb;
      | xBlock( config, {io_dir, arith_type, bitwidth, bin_pt, ... 
      |     sample_period, gw_name, latency});
      mask TypeOptions io_dir: From Processor | To Processor
      mask TypeOptions arith_type: Unsigned | Signed  (2's comp)
  arm1 : xbsIndex_r4/Slice  nbits=1  boolean_output=on  mode=Lower Bit Location + Width  bit1=0  base1=MSB of Input  bit0=2  base0=LSB of Input  dbl_ovrd=off  block_type=slice
      settings: block_version=10.1.3
  arm10 : xbsIndex_r4/Slice  nbits=1  boolean_output=on  mode=Lower Bit Location + Width  bit1=0  base1=MSB of Input  bit0=12  base0=LSB of Input  dbl_ovrd=off  block_type=slice
      settings: block_version=10.1.3
  arm11 : xbsIndex_r4/Slice  nbits=1  boolean_output=on  mode=Lower Bit Location + Width  bit1=0  base1=MSB of Input  bit0=13  base0=LSB of Input  dbl_ovrd=off  block_type=slice
      settings: block_version=10.1.3
  arm12 : xbsIndex_r4/Slice  nbits=1  boolean_output=on  mode=Lower Bit Location + Width  bit1=0  base1=MSB of Input  bit0=4  base0=LSB of Input  dbl_ovrd=off  block_type=slice
      settings: block_version=10.1.3
  arm2 : xbsIndex_r4/Slice  nbits=1  boolean_output=on  mode=Lower Bit Location + Width  bit1=0  base1=MSB of Input  bit0=3  base0=LSB of Input  dbl_ovrd=off  block_type=slice
      settings: block_version=10.1.3
  arm3 : xbsIndex_r4/Slice  nbits=1  boolean_output=on  mode=Lower Bit Location + Width  bit1=0  base1=MSB of Input  bit0=16  base0=LSB of Input  dbl_ovrd=off  block_type=slice
      settings: block_version=10.1.3
  arm4 : xbsIndex_r4/Slice  nbits=1  boolean_output=on  mode=Lower Bit Location + Width  bit1=0  base1=MSB of Input  bit0=17  base0=LSB of Input  dbl_ovrd=off  block_type=slice
      settings: block_version=10.1.3
  arm5 : xbsIndex_r4/Slice  nbits=1  boolean_output=on  mode=Lower Bit Location + Width  bit1=0  base1=MSB of Input  bit0=18  base0=LSB of Input  dbl_ovrd=off  block_type=slice
      settings: block_version=10.1.3
  arm6 : xbsIndex_r4/Slice  nbits=1  boolean_output=on  mode=Lower Bit Location + Width  bit1=0  base1=MSB of Input  bit0=19  base0=LSB of Input  dbl_ovrd=off  block_type=slice
      settings: block_version=10.1.3
  arm7 : xbsIndex_r4/Slice  nbits=1  boolean_output=on  mode=Lower Bit Location + Width  bit1=0  base1=MSB of Input  bit0=20  base0=LSB of Input  dbl_ovrd=off  block_type=slice
      settings: block_version=10.1.3
  arm8 : xbsIndex_r4/Slice  nbits=1  boolean_output=on  mode=Lower Bit Location + Width  bit1=0  base1=MSB of Input  bit0=9  base0=LSB of Input  dbl_ovrd=off  block_type=slice
      settings: block_version=10.1.3
  arm9 : xbsIndex_r4/Slice  nbits=1  boolean_output=on  mode=Lower Bit Location + Width  bit1=0  base1=MSB of Input  bit0=8  base0=LSB of Input  dbl_ovrd=off  block_type=slice
      settings: block_version=10.1.3
  auto_shutoff0 : Subsystem  mask{bits_in=8, bin_pt_in=7, clk_freq=200, acc_time=20, max_power=1/sqrt(2)}
      mask prompts: bits_in "Input bits"; bin_pt_in "Input binary point"; clk_freq "Clock frequency (MHz)"; acc_time "Window (ms)"; max_power "Max power allowed"
  auto_shutoff1 : Subsystem  mask{bits_in=8, bin_pt_in=7, clk_freq=200, acc_time=20, max_power=1/sqrt(2)}
      mask prompts: bits_in "Input bits"; bin_pt_in "Input binary point"; clk_freq "Clock frequency (MHz)"; acc_time "Window (ms)"; max_power "Max power allowed"
  board_id : xps_library/software register  Tag=xps:sw_reg  io_dir=From Processor  arith_type=Unsigned  bitwidth=32  bin_pt=0  sample_period=1  gw_name=r_128w_8k_1a_16x_r431_board_id_user_data_out
      link override r_128w_8k_1a_16x_r430_board_id_user_data_out: arith_type=Unsigned  n_bits=32  bin_pt=0  period=1
      link override r_128w_8k_1a_16x_r431_board_id_user_data_out: arith_type=Unsigned  n_bits=32  bin_pt=0  period=1
  bus_create : Subsystem  AncestorBlock=casper_library_flow_control/bus_create  mask(bus_create){inputNum=3}
      mask prompts: inputNum "Number of inputs:"
      mask init:
      | bus_create_init(gcb,...
      |     'inputNum', inputNum);
  bus_create1 : Subsystem  AncestorBlock=casper_library_flow_control/bus_create  mask(bus_create){inputNum=3}
      mask prompts: inputNum "Number of inputs:"
      mask init:
      | bus_create_init(gcb,...
      |     'inputNum', inputNum);
  bus_expand : Subsystem  AncestorBlock=casper_library_flow_control/bus_expand  mask(bus_expand){mode=divisions of arbitrary size, outputNum=2, outputWidth=[1                                     32], outputBinaryPt=[0                                      0], outputArithmeticType=[2                                      0], outputToWorkspace=off, variablePrefix=out, outputToModelAsWell=on}
      mask prompts: outputNum "Number of outputs:"; outputWidth "Output width [msb ... lsb]:"; outputBinaryPt "Output binary point position [msb ... lsb]:"; outputArithmeticType "Output arithmetic type (ufix=0, fix=1, bool=2) [msb ... lsb]:"; outputToWorkspace "Output to workspace?"; variablePrefix "Variable name prefix:"; outputToModelAsWell "Output to model as well?"
      mask help:
      | Expands a 'bus' made using a bus_create or Xilinx
      | concat block.
      | The input will be divided into the specified number
      | of outputs with the specified arithmetic types.
      | Divisions are made from most significant bit.
      mask init:
      | bus_expand_init(gcb,...
      |     'mode', mode, ...
      |     'outputNum', outputNum, ...
      |     'outputWidth', outputWidth, ...
      |     'outputBinaryPt', outputBinaryPt, ...
      |     'outputArithmeticType', outputArithmeticType, ...
      |     'outputToWorkspace', outputToWorkspace, ...
      |     'variablePrefix', variablePrefix, ...
      |     'outputToModelAsWell', outputToModelAsWell);
      settings: AttributesFormatString=2 outputs
      mask TypeOptions mode: divisions of equal size | divisions of arbitrary size
      mask Callback mode: bus_expand_callback();
      mask Callback outputWidth: bus_expand_callback();
      mask Callback outputToWorkspace: bus_expand_callback();
  bus_expand1 : Subsystem  AncestorBlock=casper_library_flow_control/bus_expand  mask(bus_expand){mode=divisions of arbitrary size, outputNum=3, outputWidth=[1                                     36                                     36], outputBinaryPt=[0                                      0                                      0], outputArithmeticType=[2                                      0                                      0], outputToWorkspace=off, variablePrefix=out, outputToModelAsWell=on}
      mask prompts: outputNum "Number of outputs:"; outputWidth "Output width [msb ... lsb]:"; outputBinaryPt "Output binary point position [msb ... lsb]:"; outputArithmeticType "Output arithmetic type (ufix=0, fix=1, bool=2) [msb ... lsb]:"; outputToWorkspace "Output to workspace?"; variablePrefix "Variable name prefix:"; outputToModelAsWell "Output to model as well?"
      mask help:
      | Expands a 'bus' made using a bus_create or Xilinx
      | concat block.
      | The input will be divided into the specified number
      | of outputs with the specified arithmetic types.
      | Divisions are made from most significant bit.
      mask init: same as r_128w_8k_1a_16x_r431/bus_expand
      settings: AttributesFormatString=3 outputs
      mask TypeOptions mode: divisions of equal size | divisions of arbitrary size
      mask Callback mode: bus_expand_callback();
      mask Callback outputWidth: bus_expand_callback();
      mask Callback outputToWorkspace: bus_expand_callback();
  bus_expand2 : Subsystem  AncestorBlock=casper_library_flow_control/bus_expand  mask(bus_expand){mode=divisions of equal size, outputNum=4, outputWidth=16, outputBinaryPt=1, outputArithmeticType=1, outputToWorkspace=off, variablePrefix=out, outputToModelAsWell=on}
      mask prompts: outputNum "Number of outputs:"; outputWidth "Output width:"; outputBinaryPt "Output binary point position:"; outputArithmeticType "Output arithmetic type (ufix=0, fix=1, bool=2):"; outputToWorkspace "Output to workspace?"; variablePrefix "Variable name prefix:"; outputToModelAsWell "Output to model as well?"
      mask help:
      | Expands a 'bus' made using a bus_create or Xilinx
      | concat block.
      | The input will be divided into the specified number
      | of outputs with the specified arithmetic types.
      | Divisions are made from most significant bit.
      mask init: same as r_128w_8k_1a_16x_r431/bus_expand
      settings: AttributesFormatString=4 outputs
      mask TypeOptions mode: divisions of equal size | divisions of arbitrary size
      mask Callback mode: bus_expand_callback();
      mask Callback outputWidth: bus_expand_callback();
      mask Callback outputToWorkspace: bus_expand_callback();
  bus_expand3 : Subsystem  AncestorBlock=casper_library_flow_control/bus_expand  mask(bus_expand){mode=divisions of arbitrary size, outputNum=3, outputWidth=[1                                     36                                     36], outputBinaryPt=[0                                      0                                      0], outputArithmeticType=[2                                      0                                      0], outputToWorkspace=off, variablePrefix=out, outputToModelAsWell=on}
      mask prompts: outputNum "Number of outputs:"; outputWidth "Output width [msb ... lsb]:"; outputBinaryPt "Output binary point position [msb ... lsb]:"; outputArithmeticType "Output arithmetic type (ufix=0, fix=1, bool=2) [msb ... lsb]:"; outputToWorkspace "Output to workspace?"; variablePrefix "Variable name prefix:"; outputToModelAsWell "Output to model as well?"
      mask help:
      | Expands a 'bus' made using a bus_create or Xilinx
      | concat block.
      | The input will be divided into the specified number
      | of outputs with the specified arithmetic types.
      | Divisions are made from most significant bit.
      mask init: same as r_128w_8k_1a_16x_r431/bus_expand
      settings: AttributesFormatString=3 outputs
      mask TypeOptions mode: divisions of equal size | divisions of arbitrary size
      mask Callback mode: bus_expand_callback();
      mask Callback outputWidth: bus_expand_callback();
      mask Callback outputToWorkspace: bus_expand_callback();
  bus_expand4 : Subsystem  AncestorBlock=casper_library_flow_control/bus_expand  mask(bus_expand){mode=divisions of equal size, outputNum=4, outputWidth=16, outputBinaryPt=1, outputArithmeticType=1, outputToWorkspace=off, variablePrefix=out, outputToModelAsWell=on}
      mask prompts: outputNum "Number of outputs:"; outputWidth "Output width:"; outputBinaryPt "Output binary point position:"; outputArithmeticType "Output arithmetic type (ufix=0, fix=1, bool=2):"; outputToWorkspace "Output to workspace?"; variablePrefix "Variable name prefix:"; outputToModelAsWell "Output to model as well?"
      mask help:
      | Expands a 'bus' made using a bus_create or Xilinx
      | concat block.
      | The input will be divided into the specified number
      | of outputs with the specified arithmetic types.
      | Divisions are made from most significant bit.
      mask init: same as r_128w_8k_1a_16x_r431/bus_expand
      settings: AttributesFormatString=4 outputs
      mask TypeOptions mode: divisions of equal size | divisions of arbitrary size
      mask Callback mode: bus_expand_callback();
      mask Callback outputWidth: bus_expand_callback();
      mask Callback outputToWorkspace: bus_expand_callback();
  bus_expand5 : Subsystem  AncestorBlock=casper_library_flow_control/bus_expand  mask(bus_expand){mode=divisions of arbitrary size, outputNum=2, outputWidth=[1                                     32], outputBinaryPt=[0                                      0], outputArithmeticType=[2                                      0], outputToWorkspace=off, variablePrefix=out, outputToModelAsWell=on}
      mask prompts: outputNum "Number of outputs:"; outputWidth "Output width [msb ... lsb]:"; outputBinaryPt "Output binary point position [msb ... lsb]:"; outputArithmeticType "Output arithmetic type (ufix=0, fix=1, bool=2) [msb ... lsb]:"; outputToWorkspace "Output to workspace?"; variablePrefix "Variable name prefix:"; outputToModelAsWell "Output to model as well?"
      mask help:
      | Expands a 'bus' made using a bus_create or Xilinx
      | concat block.
      | The input will be divided into the specified number
      | of outputs with the specified arithmetic types.
      | Divisions are made from most significant bit.
      mask init: same as r_128w_8k_1a_16x_r431/bus_expand
      settings: AttributesFormatString=2 outputs
      mask TypeOptions mode: divisions of equal size | divisions of arbitrary size
      mask Callback mode: bus_expand_callback();
      mask Callback outputWidth: bus_expand_callback();
      mask Callback outputToWorkspace: bus_expand_callback();
  bus_expand6 : Subsystem  AncestorBlock=casper_library_flow_control/bus_expand  mask(bus_expand){mode=divisions of arbitrary size, outputNum=3, outputWidth=[1                                     32                                     32], outputBinaryPt=[0                                      0                                      0], outputArithmeticType=[2                                      0                                      0], outputToWorkspace=off, variablePrefix=out, outputToModelAsWell=on}
      mask prompts: outputNum "Number of outputs:"; outputWidth "Output width [msb ... lsb]:"; outputBinaryPt "Output binary point position [msb ... lsb]:"; outputArithmeticType "Output arithmetic type (ufix=0, fix=1, bool=2) [msb ... lsb]:"; outputToWorkspace "Output to workspace?"; variablePrefix "Variable name prefix:"; outputToModelAsWell "Output to model as well?"
      mask help:
      | Expands a 'bus' made using a bus_create or Xilinx
      | concat block.
      | The input will be divided into the specified number
      | of outputs with the specified arithmetic types.
      | Divisions are made from most significant bit.
      mask init: same as r_128w_8k_1a_16x_r431/bus_expand
      settings: AttributesFormatString=3 outputs
      mask TypeOptions mode: divisions of equal size | divisions of arbitrary size
      mask Callback mode: bus_expand_callback();
      mask Callback outputWidth: bus_expand_callback();
      mask Callback outputToWorkspace: bus_expand_callback();
  calc_adc_sum_sq : Subsystem
  calc_adc_sum_sq1 : Subsystem
  cd_local_time : Subsystem
  cd_tr0 : Subsystem  mask{cnt_bits=8, time_bits=48}
      mask prompts: cnt_bits "Bits in status counters"; time_bits "No LSBs in time to compare"
  cd_tr1 : Subsystem  mask{cnt_bits=8, time_bits=48}
      mask prompts: cnt_bits "Bits in status counters"; time_bits "No LSBs in time to compare"
  clk_frequency : Subsystem  Tag=xps:sw_reg  mask{io_dir=To Processor, arith_type=Unsigned, bitwidth=32, bin_pt=0, sample_period=1, latency=0}
      link override convert: arith_type=Unsigned  n_bits=32  bin_pt=0
      mask prompts: io_dir "I/O direction"; arith_type "Data Type"; bitwidth "Data bitwidth"; bin_pt "Data binary point"; sample_period "Sample period"
      mask init:
      | gw_name = clear_name(gcb);
      | config.source = str2func('software_register_init');
      | config.toplevel = gcb;
      | xBlock( config, {io_dir, arith_type, bitwidth, bin_pt, ... 
      |     sample_period, gw_name, latency});
      mask TypeOptions io_dir: From Processor | To Processor
      mask TypeOptions arith_type: Unsigned | Signed  (2's comp)
  coarse_delay0 : xps_library/software register  Tag=xps:sw_reg  io_dir=From Processor  arith_type=Unsigned  bitwidth=32  bin_pt=0  sample_period=1  gw_name=r_128w_8k_1a_16x_r431_coarse_delay0_user_data_out
      link override r_128w_8k_1a_16x_r430_coarse_delay0_user_data_out: arith_type=Unsigned  n_bits=32  bin_pt=0  period=1
      link override r_128w_8k_1a_16x_r431_coarse_delay0_user_data_out: arith_type=Unsigned  n_bits=32  bin_pt=0  period=1
  coarse_delay1 : xps_library/software register  Tag=xps:sw_reg  io_dir=From Processor  arith_type=Unsigned  bitwidth=32  bin_pt=0  sample_period=1  gw_name=r_128w_8k_1a_16x_r431_coarse_delay1_user_data_out
      link override r_128w_8k_1a_16x_r430_coarse_delay1_user_data_out: arith_type=Unsigned  n_bits=32  bin_pt=0  period=1
      link override r_128w_8k_1a_16x_r431_coarse_delay1_user_data_out: arith_type=Unsigned  n_bits=32  bin_pt=0  period=1
  control : xps_library/software register  Tag=xps:sw_reg  io_dir=From Processor  arith_type=Unsigned  bitwidth=32  bin_pt=0  sample_period=1  gw_name=r_128w_8k_1a_16x_r431_control_user_data_out
      link override r_128w_8k_1a_16x_r430_control_user_data_out: arith_type=Unsigned  n_bits=32  bin_pt=0  period=1
      link override r_128w_8k_1a_16x_r431_control_user_data_out: arith_type=Unsigned  n_bits=32  bin_pt=0  period=1
  convert : Subsystem
  ct : Subsystem  mask{input_bits=13, output_bits=7, parallel_bits=1, which_qdr=qdr0}
      mask prompts: input_bits "Input vector length (total 2^?):"; output_bits "Output packet size (2^? samples):"; parallel_bits "Parallel Input channels per polarisation (2^?)"; which_qdr "QDR to use:"
      mask init:
      | set_param([gcb, '/qdr_ct'], 'which_qdr', which_qdr);
      mask TypeOptions which_qdr: qdr0 | qdr1
  ct_tvg : Subsystem  mask{num_channels_bits=13, channel_bits=8}
      mask prompts: num_channels_bits "Number of channels (2^?):"; channel_bits "Bits per channel:"
  decat0 : Subsystem
  decat1 : Subsystem
  decat2 : Subsystem
  decat3 : Subsystem
  delay_gen0 : Subsystem  mask{fft_len=10, phase_bits=16, max_fringe_rate=23, min_fringe_rate=38, delay_bits=16+15, delay_bin_pt=16, max_delay_rate=23, min_delay_rate=38, add_latency=1, lookup_bits=11, cd_bits=15}
      mask prompts: fft_len "FFT size (2^?)"; phase_bits "Input phase resolution (2*pi/2^? radians)"; max_fringe_rate "Max fringe update rate (1/2^? radians/sample)"; min_fringe_rate "Min (non-zero) fringe rate (1/2^? radians/sample)"; delay_bits "Input delay resolution (bits)"; delay_bin_pt "Input delay binary point"; max_delay_rate "Max delay update rate (1/2^? samples/sample)"; min_delay_rate "Min (non-zero) delay update rate (1/2^? samples/sample)"; add_latency "Add latency"; lookup_bits "DDS lookup table resolution (2*pi/2^?)"; cd_bits "Coarse delay range (2^? bits)"
  delay_gen1 : Subsystem  mask{fft_len=10, phase_bits=16, max_fringe_rate=23, min_fringe_rate=38, delay_bits=16+15, delay_bin_pt=16, max_delay_rate=23, min_delay_rate=38, add_latency=1, lookup_bits=11, cd_bits=15}
      mask prompts: fft_len "FFT size (2^?)"; phase_bits "Input phase resolution (2*pi/2^? radians)"; max_fringe_rate "Max fringe update rate (1/2^? radians/sample)"; min_fringe_rate "Min (non-zero) fringe rate (1/2^? radians/sample)"; delay_bits "Input delay resolution (bits)"; delay_bin_pt "Input delay binary point"; max_delay_rate "Max delay update rate (1/2^? samples/sample)"; min_delay_rate "Min (non-zero) delay update rate (1/2^? samples/sample)"; add_latency "Add latency"; lookup_bits "DDS lookup table resolution (2*pi/2^?)"; cd_bits "Coarse delay range (2^? bits)"
  delay_tr_status0 : Subsystem  Tag=xps:sw_reg  mask{io_dir=To Processor, arith_type=Unsigned, bitwidth=32, bin_pt=0, sample_period=1, latency=0}
      link override convert: arith_type=Unsigned  n_bits=32  bin_pt=0
      mask prompts: io_dir "I/O direction"; arith_type "Data Type"; bitwidth "Data bitwidth"; bin_pt "Data binary point"; sample_period "Sample period"
      mask init:
      | gw_name = clear_name(gcb);
      | config.source = str2func('software_register_init');
      | config.toplevel = gcb;
      | xBlock( config, {io_dir, arith_type, bitwidth, bin_pt, ... 
      |     sample_period, gw_name, latency});
      mask TypeOptions io_dir: From Processor | To Processor
      mask TypeOptions arith_type: Unsigned | Signed  (2's comp)
  delay_tr_status1 : Subsystem  Tag=xps:sw_reg  mask{io_dir=To Processor, arith_type=Unsigned, bitwidth=32, bin_pt=0, sample_period=1, latency=0}
      link override convert: arith_type=Unsigned  n_bits=32  bin_pt=0
      mask prompts: io_dir "I/O direction"; arith_type "Data Type"; bitwidth "Data bitwidth"; bin_pt "Data binary point"; sample_period "Sample period"
      mask init:
      | gw_name = clear_name(gcb);
      | config.source = str2func('software_register_init');
      | config.toplevel = gcb;
      | xBlock( config, {io_dir, arith_type, bitwidth, bin_pt, ... 
      |     sample_period, gw_name, latency});
      mask TypeOptions io_dir: From Processor | To Processor
      mask TypeOptions arith_type: Unsigned | Signed  (2's comp)
  delay_wideband_prog0 : Subsystem  AncestorBlock=casper_library/Delays/delay_wideband_prog  mask(delay_wideband_prog){max_delay=32768, n_inputs_bits=2, bram_latency=2, bram_type=Dual Port}
      mask prompts: max_delay "Max Delay (Sample Clks)"; n_inputs_bits "Number of Simultaneous Inputs(2^?)"; bram_latency "BRAM Latency"; bram_type "Select type of BRAM"
      mask init:
      | delay_wideband_prog_init(gcb,...
      |     'max_delay',max_delay,...
      |     'n_inputs_bits',n_inputs_bits,...
      |     'bram_latency',bram_latency,...
      |     'bram_type',bram_type);
      mask TypeOptions bram_type: Single Port | Dual Port
  delay_wideband_prog1 : Subsystem  AncestorBlock=casper_library/Delays/delay_wideband_prog  mask(delay_wideband_prog){max_delay=32768, n_inputs_bits=2, bram_latency=2, bram_type=Dual Port}
      mask prompts: max_delay "Max Delay (Sample Clks)"; n_inputs_bits "Number of Simultaneous Inputs(2^?)"; bram_latency "BRAM Latency"; bram_type "Select type of BRAM"
      mask init:
      | delay_wideband_prog_init(gcb,...
      |     'max_delay',max_delay,...
      |     'n_inputs_bits',n_inputs_bits,...
      |     'bram_latency',bram_latency,...
      |     'bram_type',bram_type);
      mask TypeOptions bram_type: Single Port | Dual Port
  edge_detect : Subsystem  AncestorBlock=casper_library_misc/edge_detect  mask(edge_detect){edge=Falling, polarity=Active High, x_in=[0 0.08 0.08 0.16 0.16 0.24 0.24 0.32 0.32 0.4], y_in=[1  1 -1 -1 -1 -1 -1 -1 -1 -1], x_out=[0.6 0.68 0.68 0.76 0.76 0.84 0.84 0.92 0.92 1], y_out=[-1 -1  1  1 -1 -1 -1 -1 -1 -1]}
      mask prompts: edge "Edge Type"; polarity "Output Polarity"; x_in "Input X Positions"; y_in "Input Y Positions"; x_out "Output X Positions"; y_out "Output Y Positions"
      mask help: Output is active for one-cycle after each edge of the specified type (i.e. rising, falling or both).
      mask init:
      | edge_detect_init(gcb,...
      |     'edge',edge,...
      |     'polarity',polarity,...
      |     'x_in',x_in,...
      |     'x_out',x_out,...
      |     'y_in',y_in,...
      |     'y_out',y_out);
      | 
      | x_in_num=str2num(getfield(getfield(get_param(gcb,'UserData'),'parameters'),'x_in'));
      | x_out_num=str2num(getfield(getfield(get_param(gcb,'UserData'),'parameters'),'x_out'));
      | y_in_num=str2num(getfield(getfield(get_param(gcb,'UserData'),'parameters'),'y_in'));
      | y_out_num=str2num(getfield(getfield(get_param(gcb,'UserData'),'parameters'),'y_out'));
      settings: AttributesFormatString=|
      | falling edges
      | active high
      mask Help: Output is active for one-cycle after each edge of the specified type (i.e. rising, falling, or both).  Latency is zero.
      mask TypeOptions edge: Rising | Falling | Both
      mask TypeOptions polarity: Active High | Active Low
      mask Display:
      | plot(x_in_num,0.5+y_in_num*0.2);
      | plot(x_out_num,0.5+y_out_num*0.2);
  edge_detect1 : casper_library_misc/edge_detect  edge=Rising  polarity=Active High  x_in=[0 0.08 0.08 0.16 0.16 0.24 0.24 0.32 0.32 0.4]  y_in="[-1 -1  1  1  1  1  1  1  1  1]"  x_out=[0.6 0.68 0.68 0.76 0.76 0.84 0.84 0.92 0.92 1]  y_out="[-1 -1  1  1 -1 -1 -1 -1 -1 -1]"
  edge_detect2 : Subsystem  AncestorBlock=casper_library_misc/edge_detect  mask(edge_detect){edge=Rising, polarity=Active High, x_in=[0 0.08 0.08 0.16 0.16 0.24 0.24 0.32 0.32 0.4], y_in=[-1 -1  1  1  1  1  1  1  1  1], x_out=[0.6 0.68 0.68 0.76 0.76 0.84 0.84 0.92 0.92 1], y_out=[-1 -1  1  1 -1 -1 -1 -1 -1 -1]}
      mask prompts: edge "Edge Type"; polarity "Output Polarity"; x_in "Input X Positions"; y_in "Input Y Positions"; x_out "Output X Positions"; y_out "Output Y Positions"
      mask help: Output is active for one-cycle after each edge of the specified type (i.e. rising, falling or both).
      mask init: same as r_128w_8k_1a_16x_r431/edge_detect
      settings: AttributesFormatString=|
      | rising edges
      | active high
      mask Help: Output is active for one-cycle after each edge of the specified type (i.e. rising, falling, or both).  Latency is zero.
      mask TypeOptions edge: Rising | Falling | Both
      mask TypeOptions polarity: Active High | Active Low
      mask Display:
      | plot(x_in_num,0.5+y_in_num*0.2);
      | plot(x_out_num,0.5+y_out_num*0.2);
  eq0 : Subsystem  Tag=xps:bram  AncestorBlock=xps_library/Shared BRAM  mask{arith_type=Unsigned, addr_width=12, data_width=64, reg_prim_output=on, reg_core_output=on, optimization=Minimum_Area, data_bin_pt=0, init_vals=[0:2^10-1], sample_rate=1}
      mask prompts: arith_type "Output Data Type"; addr_width "Address width"; data_width "Data Width"; reg_prim_output "Register Primitive Output"; reg_core_output "Register Core Output"; data_bin_pt "Data Binary Point"; init_vals "Initial 32-bit values (simulation only)"; sample_rate "Sample rate"
      mask init:
      | shared_bram_mask;
      mask TypeOptions arith_type: Unsigned | Signed  (2's comp)
      mask TypeOptions data_width: 8 | 16 | 32 | 64 | 128
      mask TypeOptions optimization: Minimum_Area | Low_Power
  eq1 : Subsystem  Tag=xps:bram  AncestorBlock=xps_library/Shared BRAM  mask{arith_type=Unsigned, addr_width=12, data_width=64, reg_prim_output=on, reg_core_output=on, optimization=Minimum_Area, data_bin_pt=0, init_vals=[0:2^10-1], sample_rate=1}
      mask prompts: arith_type "Output Data Type"; addr_width "Address width"; data_width "Data Width"; reg_prim_output "Register Primitive Output"; reg_core_output "Register Core Output"; data_bin_pt "Data Binary Point"; init_vals "Initial 32-bit values (simulation only)"; sample_rate "Sample rate"
      mask init:
      | shared_bram_mask;
      mask TypeOptions arith_type: Unsigned | Signed  (2's comp)
      mask TypeOptions data_width: 8 | 16 | 32 | 64 | 128
      mask TypeOptions optimization: Minimum_Area | Low_Power
  err_clear_sim3 : Constant  Value=0
  err_clear_sim4 : Constant  Value=0
  fd_fs_tvg0 : Subsystem  mask{bit_width=18, bin_pt=17, constant=1/16}
      mask prompts: bit_width "bit width"; bin_pt "binary point"
  fd_fs_tvg1 : Subsystem  mask{bit_width=18, bin_pt=17, val=1/16}
      mask prompts: bit_width "bit width"; bin_pt "binary point"; val "constant"
  fd_local_time : Subsystem
  fd_tr0 : Subsystem  mask{cnt_bits=8, time_bits=48}
      mask prompts: cnt_bits "Bits in status counters"; time_bits "No LSBs in time to compare"
  fd_tr1 : Subsystem  mask{cnt_bits=8, time_bits=48}
      mask prompts: cnt_bits "Bits in status counters"; time_bits "No LSBs in time to compare"
  fft_shift0 : xps_library/software register  Tag=xps:sw_reg  io_dir=From Processor  arith_type=Unsigned  bitwidth=32  bin_pt=0  sample_period=1  gw_name=r_128w_8k_1a_16x_r431_fft_shift0_user_data_out
      link override r_128w_8k_1a_16x_r430_fft_shift0_user_data_out: arith_type=Unsigned  n_bits=32  bin_pt=0  period=1
      link override r_128w_8k_1a_16x_r431_fft_shift0_user_data_out: arith_type=Unsigned  n_bits=32  bin_pt=0  period=1
  fft_shift1 : xps_library/software register  Tag=xps:sw_reg  io_dir=From Processor  arith_type=Unsigned  bitwidth=32  bin_pt=0  sample_period=1  gw_name=r_128w_8k_1a_16x_r431_fft_shift1_user_data_out
      link override r_128w_8k_1a_16x_r430_fft_shift1_user_data_out: arith_type=Unsigned  n_bits=32  bin_pt=0  period=1
      link override r_128w_8k_1a_16x_r431_fft_shift1_user_data_out: arith_type=Unsigned  n_bits=32  bin_pt=0  period=1
  fft_wideband_real0 : Subsystem  AncestorBlock=casper_library_ffts/fft_wideband_real  mask(fft_wideband_real){FFTSize=14, n_inputs=2, input_bit_width=18, coeff_bit_width=18, unscramble=on, add_latency=2, mult_latency=2, bram_latency=2, conv_latency=2, input_latency=0, biplex_direct_latency=0, quantization=Round  (unbiased: Even Values), overflow=Wrap, arch=Virtex5, opt_target=logic, coeffs_bit_limit=10, delays_bit_limit=10, mult_spec=1, hardcode_shifts=off, shift_schedule=, dsp48_adders=on}
      mask prompts: FFTSize "Size of FFT: (2^? pts)"; n_inputs "Number of Simultaneous Inputs: (2^?)"; input_bit_width "Input/Output Bit Width"; coeff_bit_width "Coefficient Bit Width"; unscramble "Unscramble output (ie, put channels in canonical order)"; add_latency "Add Latency"; mult_latency "Mult Latency"; bram_latency "BRAM Latency"; conv_latency "Convert Latency"; input_latency "Input Latency"; biplex_direct_latency "Latency between biplexes and fft_direct"; quantization "Quantization Behavior"; overflow "Overflow Behavior"; arch "Architecture"; opt_target "Use less"; coeffs_bit_limit "Number bits above which to store stage's coefficients in BRAM (2^? bits)"; delays_bit_limit "Number bits above which to store stage's delays in BRAM (2^? bits)"; mult_spec "Multiplier impl. (0=core, 1=embedded, 2=behavioural) (left=1st stage, or just one value)"; hardcode_shifts "Hardcode shift schedule"; shift_schedule "Shift schedule"; dsp48_adders "DSP48 adders in butterfly"
      mask help: A real-sampled wideband FFT.
      mask init:
      | fft_wideband_real_init(gcb, ...
      |     'FFTSize', FFTSize, ...
      |     'n_inputs', n_inputs, ...
      |     'input_bit_width', input_bit_width, ...
      |     'coeff_bit_width', coeff_bit_width, ...
      |     'unscramble', unscramble, ...
      |     'add_latency', add_latency, ...
      |     'mult_latency', mult_latency, ...
      |     'bram_latency', bram_latency, ...
      |     'conv_latency', conv_latency, ...
      |     'input_latency', input_latency, ...
      |     'biplex_direct_latency', biplex_direct_latency, ...
      |     'quantization', quantization, ...
      |     'overflow', overflow, ...
      |     'arch', arch, ...
      |     'opt_target', opt_target, ...
      |     'coeffs_bit_limit', coeffs_bit_limit, ...
      |     'delays_bit_limit', delays_bit_limit, ...
      |     'mult_spec', mult_spec, ...
      |     'hardcode_shifts', hardcode_shifts, ...
      |     'shift_schedule', shift_schedule, ...
      |     'dsp48_adders', dsp48_adders);
      settings: CopyFcn=fft_wideband_real_init(gcb);
      settings: AttributesFormatString=|
      | 14 stages
      | (18,18)
      | Round  (unbiased: Even Values)
      | Wrap
      mask Help: eval('xlWeb(''http://casper.berkeley.edu/wiki/Fft_wideband_real'')')
      mask TypeOptions quantization: Truncate | Round  (unbiased: +/- Inf) | Round  (unbiased: Even Values)
      mask TypeOptions overflow: Wrap | Saturate | Error
      mask TypeOptions arch: Virtex2Pro | Virtex5
      mask Callback arch: fft_callback_arch(gcb);
      mask TypeOptions opt_target: logic | multipliers
      mask Callback hardcode_shifts:
      | hardcode_shifts = get_param(gcb, 'hardcode_shifts');
      | set_param_state(gcb, 'shift_schedule', hardcode_shifts);
      mask Callback dsp48_adders: fft_callback_dsp48_adders(gcb);
  fft_wideband_real1 : Subsystem  AncestorBlock=casper_library_ffts/fft_wideband_real  mask(fft_wideband_real){FFTSize=14, n_inputs=2, input_bit_width=18, coeff_bit_width=18, unscramble=on, add_latency=2, mult_latency=2, bram_latency=2, conv_latency=2, input_latency=0, biplex_direct_latency=0, quantization=Round  (unbiased: Even Values), overflow=Wrap, arch=Virtex5, opt_target=logic, coeffs_bit_limit=10, delays_bit_limit=10, mult_spec=1, hardcode_shifts=off, shift_schedule=, dsp48_adders=on}
      mask prompts: FFTSize "Size of FFT: (2^? pts)"; n_inputs "Number of Simultaneous Inputs: (2^?)"; input_bit_width "Input/Output Bit Width"; coeff_bit_width "Coefficient Bit Width"; unscramble "Unscramble output (ie, put channels in canonical order)"; add_latency "Add Latency"; mult_latency "Mult Latency"; bram_latency "BRAM Latency"; conv_latency "Convert Latency"; input_latency "Input Latency"; biplex_direct_latency "Latency between biplexes and fft_direct"; quantization "Quantization Behavior"; overflow "Overflow Behavior"; arch "Architecture"; opt_target "Use less"; coeffs_bit_limit "Number bits above which to store stage's coefficients in BRAM (2^? bits)"; delays_bit_limit "Number bits above which to store stage's delays in BRAM (2^? bits)"; mult_spec "Multiplier impl. (0=core, 1=embedded, 2=behavioural) (left=1st stage, or just one value)"; hardcode_shifts "Hardcode shift schedule"; shift_schedule "Shift schedule"; dsp48_adders "DSP48 adders in butterfly"
      mask help: A real-sampled wideband FFT.
      mask init: same as r_128w_8k_1a_16x_r431/fft_wideband_real0
      settings: CopyFcn=fft_wideband_real_init(gcb);
      settings: AttributesFormatString=|
      | 14 stages
      | (18,18)
      | Round  (unbiased: Even Values)
      | Wrap
      mask Help: eval('xlWeb(''http://casper.berkeley.edu/wiki/Fft_wideband_real'')')
      mask TypeOptions quantization: Truncate | Round  (unbiased: +/- Inf) | Round  (unbiased: Even Values)
      mask TypeOptions overflow: Wrap | Saturate | Error
      mask TypeOptions arch: Virtex2Pro | Virtex5
      mask Callback arch: fft_callback_arch(gcb);
      mask TypeOptions opt_target: logic | multipliers
      mask Callback hardcode_shifts:
      | hardcode_shifts = get_param(gcb, 'hardcode_shifts');
      | set_param_state(gcb, 'shift_schedule', hardcode_shifts);
      mask Callback dsp48_adders: fft_callback_dsp48_adders(gcb);
  fstatus0 : Subsystem  Tag=xps:sw_reg  mask{io_dir=To Processor, arith_type=Unsigned, bitwidth=32, bin_pt=0, sample_period=1, latency=0}
      link override convert: arith_type=Unsigned  n_bits=32  bin_pt=0
      mask prompts: io_dir "I/O direction"; arith_type "Data Type"; bitwidth "Data bitwidth"; bin_pt "Data binary point"; sample_period "Sample period"
      mask init:
      | gw_name = clear_name(gcb);
      | config.source = str2func('software_register_init');
      | config.toplevel = gcb;
      | xBlock( config, {io_dir, arith_type, bitwidth, bin_pt, ... 
      |     sample_period, gw_name, latency});
      mask TypeOptions io_dir: From Processor | To Processor
      mask TypeOptions arith_type: Unsigned | Signed  (2's comp)
  fstatus1 : Subsystem  Tag=xps:sw_reg  mask{io_dir=To Processor, arith_type=Unsigned, bitwidth=32, bin_pt=0, sample_period=1, latency=0}
      link override convert: arith_type=Unsigned  n_bits=32  bin_pt=0
      mask prompts: io_dir "I/O direction"; arith_type "Data Type"; bitwidth "Data bitwidth"; bin_pt "Data binary point"; sample_period "Sample period"
      mask init:
      | gw_name = clear_name(gcb);
      | config.source = str2func('software_register_init');
      | config.toplevel = gcb;
      | xBlock( config, {io_dir, arith_type, bitwidth, bin_pt, ... 
      |     sample_period, gw_name, latency});
      mask TypeOptions io_dir: From Processor | To Processor
      mask TypeOptions arith_type: Unsigned | Signed  (2's comp)
  gbe0 : xps_library/ten_Gbe_v2  Tag=xps:tengbe_v2  flavour=cx4  slot=1  port_r1=0  port_r2_cx4=0  port_r2_sfpp=0  rx_dist_ram=on  large_frames=off  show_param=off  pre_emph_r2=0.74  pre_emph=3  post_emph_r2=0.18  rxeqmix_r2=7  swing_r2=940  swing=800  fab_en=on  fab_mac=hex2dec('123456780000')  fab_ip=192*(2^24) + 168*(2^16) + 5*(2^8) + 20*(2^0)  fab_udp=10000  fab_gate=1  cpu_rx_en=on  cpu_tx_en=on
  gbe_err : Subsystem  mask{payload_len=32}
      mask prompts: payload_len "Packet payload length in 64-bit words?"
      mask init:
      | packet_len = payload_len + 1;
      | packet_bits = ceil(log2(packet_len));
      | payload_bits = ceil(log2(payload_len));
  gbe_ip0 : xps_library/software register  Tag=xps:sw_reg  io_dir=From Processor  arith_type=Unsigned  bitwidth=32  bin_pt=0  sample_period=1  gw_name=r_128w_8k_1a_16x_r431_gbe_ip0_user_data_out
      link override r_128w_8k_1a_16x_r430_gbe_ip0_user_data_out: arith_type=Unsigned  n_bits=32  bin_pt=0  period=1
      link override r_128w_8k_1a_16x_r431_gbe_ip0_user_data_out: arith_type=Unsigned  n_bits=32  bin_pt=0  period=1
  gbe_port : xps_library/software register  Tag=xps:sw_reg  io_dir=From Processor  arith_type=Unsigned  bitwidth=32  bin_pt=0  sample_period=1  gw_name=r_128w_8k_1a_16x_r431_gbe_port_user_data_out
      link override r_128w_8k_1a_16x_r430_gbe_port_user_data_out: arith_type=Unsigned  n_bits=32  bin_pt=0  period=1
      link override r_128w_8k_1a_16x_r431_gbe_port_user_data_out: arith_type=Unsigned  n_bits=32  bin_pt=0  period=1
  gbe_tx_cnt0 : Subsystem  Tag=xps:sw_reg  mask{io_dir=To Processor, arith_type=Unsigned, bitwidth=32, bin_pt=0, sample_period=1, latency=0}
      link override convert: arith_type=Unsigned  n_bits=32  bin_pt=0
      mask prompts: io_dir "I/O direction"; arith_type "Data Type"; bitwidth "Data bitwidth"; bin_pt "Data binary point"; sample_period "Sample period"
      mask init:
      | gw_name = clear_name(gcb);
      | config.source = str2func('software_register_init');
      | config.toplevel = gcb;
      | xBlock( config, {io_dir, arith_type, bitwidth, bin_pt, ... 
      |     sample_period, gw_name, latency});
      mask TypeOptions io_dir: From Processor | To Processor
      mask TypeOptions arith_type: Unsigned | Signed  (2's comp)
  gbe_tx_err_cnt0 : Subsystem  Tag=xps:sw_reg  mask{io_dir=To Processor, arith_type=Unsigned, bitwidth=32, bin_pt=0, sample_period=1, latency=0}
      link override convert: arith_type=Unsigned  n_bits=32  bin_pt=0
      mask prompts: io_dir "I/O direction"; arith_type "Data Type"; bitwidth "Data bitwidth"; bin_pt "Data binary point"; sample_period "Sample period"
      mask init:
      | gw_name = clear_name(gcb);
      | config.source = str2func('software_register_init');
      | config.toplevel = gcb;
      | xBlock( config, {io_dir, arith_type, bitwidth, bin_pt, ... 
      |     sample_period, gw_name, latency});
      mask TypeOptions io_dir: From Processor | To Processor
      mask TypeOptions arith_type: Unsigned | Signed  (2's comp)
  gpio_tr : Subsystem  mask{cnt_bits=8, time_bits=48}
      mask prompts: cnt_bits "Bits in status counters"; time_bits "No LSBs in time to compare"
  katadc0 : Subsystem  Tag=xps:katadc  AncestorBlock=xps_library/katadc  mask(katadc){adc_brd=adc0, adc_interleave=off, bypass_auto=off, en_gain=on, adc_clk_rate=800, sample_period=1}
      mask prompts: adc_brd "ADC board"; adc_interleave "ADC interleave mode"; bypass_auto "Bypass auto config"; en_gain "Enable gain"; adc_clk_rate "ADC sampling rate (MHz)"; sample_period "Sample period"
      mask init:
      | name = gcb;
      | katadc_init(gcb, ...
      |     'name', name, ...
      |     'adc_brd', adc_brd, ...
      |     'adc_interleave', adc_interleave, ...
      |     'bypass_auto', bypass_auto, ...
      |     'en_gain', en_gain, ...
      |     'adc_clk_rate', adc_clk_rate, ...
      |     'sample_period', sample_period);
      mask TypeOptions adc_brd: adc0 | adc1
  ld_time_lsw0 : xps_library/software register  Tag=xps:sw_reg  io_dir=From Processor  arith_type=Unsigned  bitwidth=32  bin_pt=0  sample_period=1  gw_name=r_128w_8k_1a_16x_r431_ld_time_lsw0_user_data_out
      link override r_128w_8k_1a_16x_r430_ld_time_lsw0_user_data_out: arith_type=Unsigned  n_bits=32  bin_pt=0  period=1
      link override r_128w_8k_1a_16x_r431_ld_time_lsw0_user_data_out: arith_type=Unsigned  n_bits=32  bin_pt=0  period=1
  ld_time_lsw1 : xps_library/software register  Tag=xps:sw_reg  io_dir=From Processor  arith_type=Unsigned  bitwidth=32  bin_pt=0  sample_period=1  gw_name=r_128w_8k_1a_16x_r431_ld_time_lsw1_user_data_out
      link override r_128w_8k_1a_16x_r430_ld_time_lsw1_user_data_out: arith_type=Unsigned  n_bits=32  bin_pt=0  period=1
      link override r_128w_8k_1a_16x_r431_ld_time_lsw1_user_data_out: arith_type=Unsigned  n_bits=32  bin_pt=0  period=1
  ld_time_msw0 : xps_library/software register  Tag=xps:sw_reg  io_dir=From Processor  arith_type=Unsigned  bitwidth=32  bin_pt=0  sample_period=1  gw_name=r_128w_8k_1a_16x_r431_ld_time_msw0_user_data_out
      link override r_128w_8k_1a_16x_r430_ld_time_msw0_user_data_out: arith_type=Unsigned  n_bits=32  bin_pt=0  period=1
      link override r_128w_8k_1a_16x_r431_ld_time_msw0_user_data_out: arith_type=Unsigned  n_bits=32  bin_pt=0  period=1
  ld_time_msw1 : xps_library/software register  Tag=xps:sw_reg  io_dir=From Processor  arith_type=Unsigned  bitwidth=32  bin_pt=0  sample_period=1  gw_name=r_128w_8k_1a_16x_r431_ld_time_msw1_user_data_out
      link override r_128w_8k_1a_16x_r430_ld_time_msw1_user_data_out: arith_type=Unsigned  n_bits=32  bin_pt=0  period=1
      link override r_128w_8k_1a_16x_r431_ld_time_msw1_user_data_out: arith_type=Unsigned  n_bits=32  bin_pt=0  period=1
  leds : Subsystem
  man_sync1 : xbsIndex_r4/Slice  nbits=1  boolean_output=on  mode=Lower Bit Location + Width  bit1=0  base1=MSB of Input  bit0=1  base0=LSB of Input  dbl_ovrd=off  block_type=slice
      settings: block_version=10.1.3
  mcount_lsw : Subsystem  Tag=xps:sw_reg  mask{io_dir=To Processor, arith_type=Unsigned, bitwidth=32, bin_pt=0, sample_period=1, latency=0}
      link override convert: arith_type=Unsigned  n_bits=32  bin_pt=0
      mask prompts: io_dir "I/O direction"; arith_type "Data Type"; bitwidth "Data bitwidth"; bin_pt "Data binary point"; sample_period "Sample period"
      mask init:
      | gw_name = clear_name(gcb);
      | config.source = str2func('software_register_init');
      | config.toplevel = gcb;
      | xBlock( config, {io_dir, arith_type, bitwidth, bin_pt, ... 
      |     sample_period, gw_name, latency});
      mask TypeOptions io_dir: From Processor | To Processor
      mask TypeOptions arith_type: Unsigned | Signed  (2's comp)
  mcount_msw : Subsystem  Tag=xps:sw_reg  mask{io_dir=To Processor, arith_type=Unsigned, bitwidth=32, bin_pt=0, sample_period=1, latency=0}
      link override convert: arith_type=Unsigned  n_bits=32  bin_pt=0
      mask prompts: io_dir "I/O direction"; arith_type "Data Type"; bitwidth "Data bitwidth"; bin_pt "Data binary point"; sample_period "Sample period"
      mask init:
      | gw_name = clear_name(gcb);
      | config.source = str2func('software_register_init');
      | config.toplevel = gcb;
      | xBlock( config, {io_dir, arith_type, bitwidth, bin_pt, ... 
      |     sample_period, gw_name, latency});
      mask TypeOptions io_dir: From Processor | To Processor
      mask TypeOptions arith_type: Unsigned | Signed  (2's comp)
  packetiser : Subsystem  mask{payload_bits=5, xengine_bits=4, fft_bits=13}
      mask prompts: payload_bits "Payload length in 64bit words (2^?)"; xengine_bits "Number of x-engines (2^?)"; fft_bits "Number of frequencies (2^?)"
      mask help: Package 32 bit data into 64 bits and identify data as coming from antenna 0 or 1
  pfb_fir_real : Subsystem  AncestorBlock=casper_library_pfbs/pfb_fir_real  mask(pfb_fir_real){PFBSize=14, TotalTaps=4, WindowType=hamming, n_inputs=2, MakeBiplex=on, BitWidthIn=8, BitWidthOut=18, CoeffBitWidth=18, CoeffDistMem=off, add_latency=1, mult_latency=3, bram_latency=2, fan_latency=1, conv_latency=1, quantization=Round  (unbiased: Even Values), fwidth=1, mult_spec=1, adder_folding=on, adder_imp=Behavioral, coeffs_share=on}
      mask prompts: PFBSize "Size of PFB: (2^? pnts)"; TotalTaps "Total Number of Taps:"; WindowType "Windowing Function:"; n_inputs "Number of Simultaneous Inputs: (2^?)"; MakeBiplex "Make Biplex?"; BitWidthIn "Input Bitwidth:"; BitWidthOut "Output Bitwidth:"; CoeffBitWidth "Coefficient Bitwidth:"; CoeffDistMem "Use Distributed Memory for Coeffs"; add_latency "Add Latency"; mult_latency "Mult Latency"; bram_latency "BRAM Latency"; fan_latency "Fanout latency"; conv_latency "Convert latency"; quantization "Quantization Behavior"; fwidth "Bin Width Scaling (normal=1)"; mult_spec "Multiplier specification (0=core, 1=embedded, 2=behavioural) (left=1st tap, or just one value)"; adder_folding "Fold adders into DSPs"; adder_imp "Adder implementation"; coeffs_share "Share coefficients between polarisations (use less BRAM)?"
      mask help:
      | Fold adders into DSPs: Causes adders to be absorbed into DSP blocks (supported in Virtex5)
      | Adder implementation: Cores using Fabric or DSP48 or behavioral HDL
      mask init:
      | pfb_fir_real_init(gcb, ...
      |     'PFBSize', PFBSize, ...
      |     'TotalTaps', TotalTaps, ...
      |     'WindowType', WindowType, ...
      |     'n_inputs', n_inputs, ...
      |     'MakeBiplex', MakeBiplex, ...
      |     'BitWidthIn', BitWidthIn, ...
      |     'BitWidthOut', BitWidthOut, ...
      |     'CoeffBitWidth', CoeffBitWidth, ...
      |     'CoeffDistMem', CoeffDistMem, ...
      |     'add_latency', add_latency, ...
      |     'mult_latency', mult_latency, ...
      |     'bram_latency', bram_latency, ...
      |     'fan_latency', fan_latency, ...
      |     'conv_latency', conv_latency, ...
      |     'quantization', quantization, ...
      |     'fwidth', fwidth, ...
      |     'mult_spec', mult_spec, ...
      |     'adder_folding', adder_folding, ...
      |     'adder_imp', adder_imp, ...
      |     'coeffs_share', coeffs_share);
      settings: AttributesFormatString=taps=4, add_latency=1
      mask Help: eval('xlWeb(''http://casper.berkeley.edu/wiki/Pfb_fir_real'')')
      mask Callback TotalTaps:
      | %num_taps = eval(get_param(gcb, 'TotalTaps'));
      | %old_vec = eval(get_param(gcb, 'mult_spec'));=-0l
      | 
      | %vec = 2.*ones(1,num_taps);
      | %old_size = length(old_vec);
      | 
      | %if(old_size <= num_taps),
      | %    new_size = old_size;
      | %else,
      | %    new_size = num_taps;
      | %end
      | 
      | %for n = 1:new_size, vec(n) = old_vec(n); end
      | %set_param(gcb, 'mult_spec', mat2str(vec));
      mask TypeOptions WindowType: bartlett | barthannwin | blackman | blackmanharris | bohamwin | chebwin | flattopwin | gausswin | hamming | hann | kaiser | nuttallwin | parzenwin | rectwin | tukeywin | triang | userwindow
      mask TypeOptions quantization: Truncate | Round  (unbiased: +/- Inf) | Round  (unbiased: Even Values)
      mask TypeOptions adder_imp: Behavioral | Fabric | DSP48
  pkt_cont_tvg0 : Subsystem  mask{p_bits=5, fft_bits=13, x_bits=4}
      mask prompts: p_bits "packet size (2^? 64 bit words)"; fft_bits "Number of channels (2^?)"; x_bits "n_x_engines (2^?)"
  pol_pack0 : Subsystem
  pol_pack1 : Subsystem
  posedge{1..3,23..24} (5 alike) : casper_library_misc/posedge  Tag=Rising Edge Detector
  pps_count : Subsystem  Tag=xps:sw_reg  mask{io_dir=To Processor, arith_type=Unsigned, bitwidth=32, bin_pt=0, sample_period=1, latency=0}
      link override convert: arith_type=Unsigned  n_bits=32  bin_pt=0
      mask prompts: io_dir "I/O direction"; arith_type "Data Type"; bitwidth "Data bitwidth"; bin_pt "Data binary point"; sample_period "Sample period"
      mask init:
      | gw_name = clear_name(gcb);
      | config.source = str2func('software_register_init');
      | config.toplevel = gcb;
      | xBlock( config, {io_dir, arith_type, bitwidth, bin_pt, ... 
      |     sample_period, gw_name, latency});
      mask TypeOptions io_dir: From Processor | To Processor
      mask TypeOptions arith_type: Unsigned | Signed  (2's comp)
  quant0 : Subsystem  mask{channel_bits=13, din_bit_width=18, din_bin_pt=17, coeff_bit_width=16, coeff_bin_pt=1, dout_bit_width=4, dout_bin_pt=3, init_val=4, overflow=Saturate, quantization=Round  (unbiased: even values), conv_latency=2, add_latency=1, mult_latency=2, bram_latency=2}
      mask prompts: channel_bits "Number channels (2^?)"; din_bit_width "Data input bit width"; din_bin_pt "Data input binary point"; coeff_bit_width "Coefficient bit width"; coeff_bin_pt "Coefficient binary point"; dout_bit_width "Data out bit width"; dout_bin_pt "Data out binary point"; init_val "Initial value"; overflow "Overflow behaviour"; quantization "Quantization Behaviour"; conv_latency "Conversion latency"; add_latency "Adder latency"; mult_latency "Multiplier latency"; bram_latency "BRAM latency"
      mask init:
      | blk = gcb;
      | set_param([blk,'/convert_of0'], ...
      |     'bit_width_i', num2str(din_bit_width+coeff_bit_width+1), ...
      |     'binary_point_i', num2str(din_bin_pt+coeff_bin_pt), ...
      |     'bit_width_o', num2str(dout_bit_width), 'binary_point_o', num2str(dout_bin_pt), ...
      |     'latency', num2str(conv_latency), 'overflow', overflow, ...
      |     'quantization', quantization);
      | set_param([blk,'/convert_of1'], ...
      |     'bit_width_i', num2str(din_bit_width+coeff_bit_width+1), ...
      |     'binary_point_i', num2str(din_bin_pt+coeff_bin_pt), ...
      |     'bit_width_o', num2str(dout_bit_width), 'binary_point_o', num2str(dout_bin_pt), ...
      |     'latency', num2str(conv_latency), 'overflow', overflow, ...
      |     'quantization', quantization);
      | set_param([blk,'/convert_of2'], ...
      |     'bit_width_i', num2str(din_bit_width+coeff_bit_width+1), ...
      |     'binary_point_i', num2str(din_bin_pt+coeff_bin_pt), ...
      |     'bit_width_o', num2str(dout_bit_width), 'binary_point_o', num2str(dout_bin_pt), ...
      |     'latency', num2str(conv_latency), 'overflow', overflow, ...
      |     'quantization', quantization);
      | set_param([blk,'/convert_of3'], ...
      |     'bit_width_i', num2str(din_bit_width+coeff_bit_width+1), ...
      |     'binary_point_i', num2str(din_bin_pt+coeff_bin_pt), ...
      |     'bit_width_o', num2str(dout_bit_width), 'binary_point_o', num2str(dout_bin_pt), ...
      |     'latency', num2str(conv_latency), 'overflow', overflow, ...
      |     'quantization', quantization);
      mask TypeOptions overflow: Wrap | Saturate | Error
      mask TypeOptions quantization: Truncate | Round  (unbiased: +/- Inf) | Round  (unbiased: even values)
  quant1 : Subsystem  mask{channel_bits=13, din_bit_width=18, din_bin_pt=17, coeff_bit_width=16, coeff_bin_pt=1, dout_bit_width=4, dout_bin_pt=3, init_val=4, overflow=Saturate, quantization=Round  (unbiased: even values), conv_latency=2, add_latency=1, mult_latency=2, bram_latency=2}
      mask prompts: channel_bits "Number channels (2^?)"; din_bit_width "Data input bit width"; din_bin_pt "Data input binary point"; coeff_bit_width "Coefficient bit width"; coeff_bin_pt "Coefficient binary point"; dout_bit_width "Data out bit width"; dout_bin_pt "Data out binary point"; init_val "Initial value"; overflow "Overflow behaviour"; quantization "Quantization Behaviour"; conv_latency "Conversion latency"; add_latency "Adder latency"; mult_latency "Multiplier latency"; bram_latency "BRAM latency"
      mask init: same as r_128w_8k_1a_16x_r431/quant0
      mask TypeOptions overflow: Wrap | Saturate | Error
      mask TypeOptions quantization: Truncate | Round  (unbiased: +/- Inf) | Round  (unbiased: even values)
  rcs : Subsystem  AncestorBlock=casper_library_misc/rcs  mask(rcs){app_src=timestamp, lib_src=git, user_val=430}
      mask prompts: app_src "Application revision info to capture"; lib_src "CASPER libraries revision info to capture"; user_val "User specified value"
      mask help:
      | Embeds revision control information for the user design and libraries.
      | On failure to locate specified revision information, falls back to
      | timestamps (current time for libraries).
      | A user specified value is also stored.
      mask init:
      | rcs_init(gcb, ...
      |     'app_src', app_src, ...
      |     'lib_src', lib_src);
      mask TypeOptions app_src: timestamp | git | svn
      mask TypeOptions lib_src: timestamp | git | svn
  scopes : Subsystem
  snap_gbe_tx0 : Subsystem  Tag=casper:snapshot  AncestorBlock=casper_library_scopes/snapshot  mask(snapshot){storage=bram, dram_dimm=1, dram_clock=200, nsamples=8, data_width=128, offset=on, circap=off, value=off, use_dsp48=off}
      mask prompts: storage "Storage medium"; dram_dimm "DRAM dimm"; dram_clock "DRAM clock rate"; nsamples "Number of Samples (2^?)"; data_width "Data width"; offset "Start delay support"; circap "Circular capture support"; value "Extra value capture support"; use_dsp48 "Use DSP48s to implement counters"
      mask help:
      | Standard snap block, but with the following optional extras;
      |  1) Optionally delay the fabric trigger by a user-specified number of valids.
      |  2) Capture continuously after a trigger until a stop pulse is received. Data is captured into BRAM continuously, with old data being overwritten until a stop command is received. Then stop capturing when memory is filled. This enables you to get some data before and some data after the stop pulse. Use the 'tr_en_cnt' register to determine where you are in your vector. 'Addr' register's MSb now indicates 'busy capturing'.
      |  3) Optionally capture a value on an input port to a register at the same time as the first data sample.
      |  4) Implement counters using DSP48Es to save resources.
      mask init: same as r_128w_8k_1a_16x_r431/adc_snap0
      mask TypeOptions storage: bram | dram
      mask Callback storage: snapshot_callback();
      mask TypeOptions dram_dimm: 1 | 2 | 3 | 4
      mask TypeOptions dram_clock: 200 | 250 | 266 | 300 | 333
      mask TypeOptions data_width: 8 | 16 | 32 | 64 | 128
  timing : Subsystem  mask{reset_period=1, sync_gen_bits=32}
      mask prompts: reset_period "Master reset time (sync pulses)"; sync_gen_bits "Size of sync generator counter (bits)"
  trig0 : Subsystem  mask{mult_latency=3}
      mask prompts: mult_latency "Multiplier latency"
  trig1 : Subsystem  mask{mult_latency=3}
      mask prompts: mult_latency "Multiplier latency"
  trig_level : xps_library/software register  Tag=xps:sw_reg  io_dir=From Processor  arith_type=Unsigned  bitwidth=32  bin_pt=0  sample_period=1  gw_name=r_128w_8k_1a_16x_r431_trig_level_user_data_out
      link override r_128w_8k_1a_16x_r430_trig_level_user_data_out: arith_type=Unsigned  n_bits=32  bin_pt=0  period=1
      link override r_128w_8k_1a_16x_r431_trig_level_user_data_out: arith_type=Unsigned  n_bits=32  bin_pt=0  period=1
  tvg_tr : Subsystem  mask{cnt_bits=8, time_bits=48}
      mask prompts: cnt_bits "Bits in status counters"; time_bits "No LSBs in time to compare"
  unpack0 : Subsystem
  unpack1 : Subsystem
  xaui_pack0 : Subsystem  mask{payload_len=32, xeng_bits=4, chan_bits=13, skip_xeng_bits=1}
      mask prompts: payload_len "Payload Length (in 64 bit words)"; xeng_bits "Number of X engines (2^?)"; chan_bits "Number of Frequency channels (2^?)"; skip_xeng_bits "X engines per IP address (2^?)"
      mask help: Packetizes data coming in over a XAUI interface. A packet consists of a 64 bit header (48 bits of "mcnt" and 16 bits of antenna), followed by 64 x "payload" bits of payload. "Mcnt" (master count) is a counter which keeps track of how many packets have been transmitted since the last "mrst".
      mask init:
      | packet_len = payload_len + 1;
      | packet_bits = ceil(log2(packet_len));
      | payload_bits = ceil(log2(payload_len));
  wires:
  [adc_sync0] -> Logical3/2
  timing/2(sync) -> [sync]
  Logical3/1 -> timing/4(pps_in), [pps]
  Concat/1 -> timing/2(data_in)
  Constant9/1 -> fft_shift0/1
  fft_shift0/1 -> Slice6/1
  a0p0_1st_shift/2(dout1) -> fft_wideband_real0/3(in0)
  a0p0_1st_shift/3(dout2) -> fft_wideband_real0/4(in1)
  a0p0_1st_shift/4(dout3) -> fft_wideband_real0/5(in2)
  a0p0_1st_shift/5(dout4) -> fft_wideband_real0/6(in3)
  Slice6/1 -> fft_wideband_real0/2(shift)
  a0p0_1st_shift/1(sync_out) -> fft_wideband_real0/1(sync)
  fft_wideband_real0/1(sync_out) -> fd_local_time/2(sync), Delay20/1
  fft_wideband_real0/4(of) -> [fft_or0]
  a0p1_1st_shift/2(dout1) -> fft_wideband_real1/3(in0)
  a0p1_1st_shift/3(dout2) -> fft_wideband_real1/4(in1)
  a0p1_1st_shift/4(dout3) -> fft_wideband_real1/5(in2)
  a0p1_1st_shift/5(dout4) -> fft_wideband_real1/6(in3)
  a0p1_1st_shift/1(sync_out) -> fft_wideband_real1/1(sync)
  unpack0/1(Out1) -> delay_wideband_prog0/4(data_in1)
  unpack0/2(Out2) -> delay_wideband_prog0/5(data_in2)
  unpack0/3(Out3) -> delay_wideband_prog0/6(data_in3)
  unpack0/4(Out4) -> delay_wideband_prog0/7(data_in4)
  delay_wideband_prog0/1(sync_out) -> pfb_fir_real/1(sync)
  delay_wideband_prog0/2(data_out1) -> pfb_fir_real/2(pol1_in1)
  delay_wideband_prog0/3(data_out2) -> pfb_fir_real/3(pol1_in2)
  delay_wideband_prog0/4(data_out3) -> pfb_fir_real/4(pol1_in3)
  delay_wideband_prog0/5(data_out4) -> pfb_fir_real/5(pol1_in4)
  quant0/2(dout0) -> Concat7/1
  quant0/3(dout1) -> Concat7/2
  quant0/1(sync_out) -> [quant0_sync]
  quant0/4(of) -> [quant_or0]
  Concat7/1 -> [quant0_data]
  timing/1(armed) -> Logical14/2, [armed]
  Logical14/1 -> [mrst]
  [mrst] -> cd_local_time/1(reset)
  [sync] -> cd_local_time/2(sync)
  cd_local_time/1(time) -> [cd_local_time]
  [sys_rst] -> Logical14/1
  [man_sync] -> Logical3/1
  [arm] -> timing/1(arm)
  Constant2/1 -> timing/3(sync_period)
  pfb_fir_real/2(pol1_out1) -> a0p0_1st_shift/2(din1)
  pfb_fir_real/3(pol1_out2) -> a0p0_1st_shift/3(din2)
  pfb_fir_real/4(pol1_out3) -> a0p0_1st_shift/4(din3)
  pfb_fir_real/5(pol1_out4) -> a0p0_1st_shift/5(din4)
  pfb_fir_real/1(sync_out) -> a0p1_1st_shift/1(sync_in), a0p0_1st_shift/1(sync_in)
  Constant33/1 -> ld_time_msw0/1
  Constant29/1 -> ld_time_lsw0/1
  ld_time_msw0/1 -> Slice73/1, Slice7/1
  Slice73/1 -> Concat9/1
  ld_time_lsw0/1 -> Concat9/2
  fstatus0/1(sim_reg_out) -> Terminator9/1
  Constant18/1 -> control/1
  control/1 -> Delay6/1
  Delay6/1 -> Slice78/1, man_sync1/1, arm1/1, arm2/1, arm8/1, arm10/1, arm6/1, arm7/1, arm5/1, arm4/1, arm3/1, arm11/1, arm9/1, arm12/1
  Slice78/1 -> [sys_rst]
  man_sync1/1 -> posedge1/1
  posedge1/1 -> [man_sync]
  arm1/1 -> posedge24/1
  posedge24/1 -> [arm]
  arm2/1 -> posedge23/1
  posedge23/1 -> [clr_status]
  Counter1/1 -> Register19/1
  Register19/1 -> clk_frequency/1(reg_out), Relational/1, Relational1/1
  clk_frequency/1(sim_reg_out) -> Terminator10/1
  pps_count/1(sim_reg_out) -> Terminator11/1
  [mrst] -> Counter3/1
  [cd_local_time] -> Delay7/1
  mcount_msw/1(sim_reg_out) -> Terminator12/1
  mcount_lsw/1(sim_reg_out) -> Terminator13/1
  Slice/1 -> mcount_lsw/1(reg_out)
  Slice1/1 -> mcount_msw/1(reg_out)
  fstatus1/1(sim_reg_out) -> Terminator2/1
  Constant32/1 -> coarse_delay0/1
  Constant8/1 -> a0_fd0/1
  Constant4/1 -> a1_fd0/1
  a0_fd0/1 -> Slice3/1, Slice2/1
  Slice4/1 -> Concat22/4
  Slice5/1 -> Concat22/5
  cd_tr0/1(arm_count) -> Terminator14/1
  Constant27/1 -> adc_ctrl0/1
  adc_ctrl0/1 -> Slice29/1, Slice30/1
  Logical/1 -> edge_detect1/1
  edge_detect1/1 -> [adc_sync0]
  [mrst] -> fd_local_time/1(reset)
  fd_local_time/1(time) -> tvg_tr/4(current_time), Delay24/1
  [armed] -> Concat21/1
  Counter3/1 -> Concat21/2
  Concat21/1 -> pps_count/1(reg_out)
  Constant40/1 -> fft_shift1/1
  fft_shift1/1 -> Slice26/1
  Slice26/1 -> fft_wideband_real1/2(shift)
  calc_adc_sum_sq/1(sum_sq) -> Delay8/1
  decat0/1(Out1) -> calc_adc_sum_sq/1(In1)
  decat0/2(Out2) -> calc_adc_sum_sq/2(In2)
  decat0/3(Out3) -> calc_adc_sum_sq/3(In3)
  decat0/4(Out4) -> calc_adc_sum_sq/4(In4)
  [adc0] -> decat0/1(In1)
  adc_sum_sq0/1(sim_reg_out) -> Terminator/1
  [adc1] -> decat1/1(In1)
  Constant48/1 -> adc_ctrl1/1
  adc_ctrl1/1 -> Slice34/1, Slice33/1
  calc_adc_sum_sq1/1(sum_sq) -> Delay12/1
  decat1/1(Out1) -> calc_adc_sum_sq1/1(In1)
  decat1/2(Out2) -> calc_adc_sum_sq1/2(In2)
  decat1/3(Out3) -> calc_adc_sum_sq1/3(In3)
  decat1/4(Out4) -> calc_adc_sum_sq1/4(In4)
  adc_sum_sq1/1(sim_reg_out) -> Terminator25/1
  Constant3/1 -> board_id/1
  board_id/1 -> [board_id]
  arm3/1 -> posedge2/1
  posedge2/1 -> [tvg_en]
  arm4/1 -> [ct_tvg]
  arm5/1 -> [packetiser_tvg]
  arm6/1 -> [fd_fs_tvg]
  [clr_status] -> Subsystem7/1(clr)
  [xaui_ldn0] -> Subsystem7/2(xuai_ldn)
  [xaui_of0] -> Subsystem7/3(xaui_of)
  [ct_err0] -> Subsystem7/4(ct_err)
  [adc_or0] -> Subsystem7/5(adc_or)
  [fft_or0] -> Subsystem7/6(fft_or)
  [quant_or0] -> Subsystem7/7(quant_or)
  bus_expand1/1(msb_out3) -> Counter8/1, Delay13/1
  Counter8/1 -> eq0/1(addr)
  Constant41/1 -> eq0/2(data_in)
  Constant46/1 -> eq0/3(we)
  arm7/1 -> [adc_tvg]
  pol_pack0/1(Out1) -> [adc0]
  pol_pack1/1(Out1) -> [adc1]
  coarse_delay0/1 -> Slice38/1
  Slice2/1 -> Concat22/1
  Slice3/1 -> Concat22/2
  [cd_val1] -> Slice22/1, Slice20/1, Slice23/1, Slice24/1, Slice21/1
  delay_gen0/1(sync_out) -> delay_wideband_prog0/1(sync)
  delay_gen0/2(en_out) -> delay_wideband_prog0/3(en)
  delay_gen0/3(cd_o) -> delay_wideband_prog0/2(delay)
  delay_gen0/4(phase_out) -> Terminator35/1
  delay_gen0/5(slope_out) -> Terminator36/1
  delay_gen0/7(idx_d0) -> Terminator37/1
  delay_gen0/8(d1) -> Terminator38/1
  delay_gen0/9(idx_d1) -> Terminator39/1
  delay_gen1/9(idx_d1) -> Terminator44/1
  delay_gen1/8(d1) -> Terminator43/1
  delay_gen1/7(idx_d0) -> Terminator42/1
  delay_gen1/1(sync_out) -> delay_wideband_prog1/1(sync)
  delay_gen1/2(en_out) -> delay_wideband_prog1/3(en)
  delay_gen1/3(cd_o) -> delay_wideband_prog1/2(delay)
  delay_gen1/4(phase_out) -> Terminator40/1
  delay_gen1/5(slope_out) -> Terminator41/1
  delay_gen1/6(d0) -> unpack1/1(In1)
  unpack1/1(Out1) -> delay_wideband_prog1/4(data_in1)
  unpack1/2(Out2) -> delay_wideband_prog1/5(data_in2)
  unpack1/3(Out3) -> delay_wideband_prog1/6(data_in3)
  unpack1/4(Out4) -> delay_wideband_prog1/7(data_in4)
  delay_gen0/6(d0) -> unpack0/1(In1)
  [mrst] -> packetiser/4(mrst_in)
  ct/4(ct_err) -> [ct_err0]
  X-engine reorder/1(sync_out) -> Recombine channels/1(sync_in)
  X-engine reorder/2(out0) -> Recombine channels/2(channel0)
  X-engine reorder/3(out1) -> Recombine channels/3(channel1)
  Recombine channels/1(sync_out) -> ct/1(sync)
  Recombine channels/2(p0) -> ct/2(p0)
  Recombine channels/3(p1) -> ct/3(p1)
  ct_tvg/1(sync_out) -> Split channels/1(sync_in)
  ct_tvg/2(p0) -> Split channels/2(p0)
  Split channels/1(sync_out) -> X-engine reorder/1(sync)
  ct_tvg/3(p1) -> Split channels/3(p1)
  Split channels/2(even) -> X-engine reorder/2(data0)
  Split channels/3(odd) -> X-engine reorder/3(data1)
  [board_id] -> packetiser/5(ant_base)
  [quant0_sync] -> ct_tvg/2(sync_in)
  [quant0_data] -> ct_tvg/3(p0_in)
  [quant1_data] -> ct_tvg/4(p1_in)
  [ct_tvg] -> Register/1
  [tvg_en] -> Register/2
  Register/1 -> ct_tvg/1(enable)
  fft_wideband_real0/2(out0) -> Delay22/1
  fft_wideband_real0/3(out1) -> Delay21/1
  fft_wideband_real1/1(sync_out) -> Delay25/1
  fft_wideband_real1/2(out0) -> Delay26/1
  fft_wideband_real1/3(out1) -> Delay27/1
  ct/1(sync_out) -> pkt_cont_tvg0/2(sync)
  ct/2(data_valid) -> pkt_cont_tvg0/3(dv)
  pkt_cont_tvg0/1(sync_out) -> packetiser/1(sync_in)
  pkt_cont_tvg0/2(dv_out) -> packetiser/2(data_valid)
  pkt_cont_tvg0/3(dout) -> packetiser/3(data_in)
  [tvg_en] -> Register1/2
  [packetiser_tvg] -> Register1/1
  Register1/1 -> pkt_cont_tvg0/1(use_tvg)
  Register2/1 -> fd_fs_tvg0/3(use_tvg), fd_fs_tvg1/1(use_tvg)
  katadc0/5(or0) -> [adc_or0]
  katadc0/1(data0_0) -> pol_pack0/1(In1)
  katadc0/2(data0_1) -> pol_pack0/2(In2)
  katadc0/3(data0_2) -> pol_pack0/3(In3)
  katadc0/4(data0_3) -> pol_pack0/4(In4)
  katadc0/6(data1_0) -> pol_pack1/1(In1)
  katadc0/7(data1_1) -> pol_pack1/2(In2)
  katadc0/8(data1_2) -> pol_pack1/3(In3)
  katadc0/9(data1_3) -> pol_pack1/4(In4)
  katadc0/10(or1) -> [adc_or1]
  katadc0/15(data_valid) -> Terminator1/1
  Pulse Generator2/1 -> katadc0/1(sim_data0)
  Pulse Generator/1 -> katadc0/2(sim_data1)
  Pulse Generator1/1 -> katadc0/3(sim_sync)
  Constant/1 -> katadc0/4(sim_data_valid)
  xaui_pack0/6(sync) -> Delay31/1(d)
  xaui_pack0/7(mrst) -> Delay34/1(d)
  xaui_pack0/5(discard) -> Delay33/1(d)
  [gbe_base_ip] -> xaui_pack0/5(base_ip)
  xaui_pack0/1(dout) -> Delay9/1(d)
  xaui_pack0/2(valid_out) -> Delay23/1(d)
  xaui_pack0/3(dest_ip) -> Delay10/1(d)
  xaui_pack0/4(eof) -> Delay11/1(d)
  Delay1/1(q) -> xaui_pack0/1(din)
  Delay3/1(q) -> xaui_pack0/2(oob)
  Delay4/1(q) -> xaui_pack0/3(valid_in)
  Delay5/1(q) -> xaui_pack0/4(linkdown_in)
  Delay31/1(q) -> [xaui_sync]
  Delay33/1(q) -> [xaui_pkt_err]
  Delay34/1(q) -> [xaui_mrst]
  [gbe_enable] -> Logical1/2
  [gbe_up] -> Subsystem3/5(link_up)
  [gbe_tx] -> Subsystem3/6(led_tx)
  [gbe_txd] -> Subsystem3/1(data_in)
  [gbe_txvld] -> Subsystem3/2(valid_in)
  [gbe_txip] -> Subsystem3/3(ip_in)
  [gbe_txeof] -> Subsystem3/4(eof_in)
  xaui_pack0/8(hdr) -> Terminator8/1
  xaui_pack0/9(hdr_valid) -> Terminator7/1
  [xaui_data] -> Delay1/1(d)
  [xaui_oob] -> Delay3/1(d)
  [xaui_valid] -> Delay4/1(d)
  [xaui_link_dn] -> Delay5/1(d)
  Delay9/1(q) -> [xaui_pkt_data]
  Delay23/1(q) -> [xaui_pkt_valid]
  Delay10/1(q) -> [xaui_pkt_ip]
  Delay11/1(q) -> [xaui_pkt_eof]
  [xaui_pkt_valid] -> Logical1/1
  Logical2/1 -> [gbe_rst_int]
  [gbe_rst] -> Logical2/2
  Constant20/1 -> Logical2/1
  Logical1/1 -> [gbe_txvld]
  [xaui_pkt_data] -> [gbe_txd]
  [xaui_pkt_ip] -> [gbe_txip]
  [xaui_pkt_eof] -> [gbe_txeof]
  [xaui_pkt_err] -> [gbe_tx_discard]
  [gbe_tx_full] -> Subsystem3/7(tx_full)
  [gbe_tx_over] -> Subsystem3/8(tx_over)
  [gbe_rst_int] -> gbe0/1
  [gbe_txd] -> gbe0/2
  [gbe_txvld] -> gbe0/3
  [gbe_txip] -> gbe0/4
  [gbe_txport] -> gbe0/5
  [gbe_txeof] -> gbe0/6
  [gbe_rxack] -> gbe0/7
  Constant5/1 -> [gbe_rxack]
  [gbe_rxack] -> gbe0/8
  gbe0/1 -> [gbe_up], Inverter/1
  gbe0/2 -> [gbe_rx]
  gbe0/3 -> [gbe_tx]
  gbe0/4 -> [gbe_tx_full]
  gbe0/5 -> [gbe_tx_over], [xaui_of0]
  gbe0/12 -> [gbe_rx_over]
  gbe0/11 -> [gbe_rx_bad]
  gbe0/6 -> [gbe_rxdata]
  gbe0/7 -> [gbe_rxvld]
  gbe0/8 -> [gbe_rxip]
  gbe0/9 -> [gbe_rxport]
  gbe0/10 -> [gbe_rxeof]
  err_clear_sim4/1 -> gbe_port/1
  gbe_port/1 -> Delay71/1(d)
  err_clear_sim3/1 -> gbe_ip0/1
  gbe_ip0/1 -> Delay72/1(d)
  Delay71/1(q) -> [gbe_txport]
  Delay72/1(q) -> [gbe_base_ip]
  packetiser/1(data_out) -> [xaui_data]
  packetiser/2(oob) -> [xaui_oob]
  packetiser/3(valid_out) -> [xaui_valid]
  Constant7/1 -> [xaui_link_dn]
  arm8/1 -> Delay100/1(d)
  arm9/1 -> Delay2/1(d)
  Delay100/1(q) -> [gbe_enable]
  Delay2/1(q) -> [gbe_rst]
  Inverter/1 -> [xaui_ldn0]
  gbe_err/1(tx_cnt) -> Delay14/1(d)
  [clr_status] -> gbe_err/1(rst)
  gbe_err/2(err_cnt) -> Delay64/1(d)
  gbe_tx_err_cnt0/1(sim_reg_out) -> Terminator4/1
  Delay64/1(q) -> gbe_tx_err_cnt0/1(reg_out)
  [gbe_tx_discard] -> gbe_err/2(discard)
  [gbe_txeof] -> gbe_err/3(eof)
  [gbe_txvld] -> gbe_err/4(valid)
  arm10/1 -> [fancy_en]
  [cd_val0] -> Slice16/1, Slice19/1, Slice18/1, Slice15/1, Slice17/1
  [cd_en0] -> delay_gen0/2(en)
  Slice16/1 -> delay_gen0/3(phase)
  Slice19/1 -> delay_gen0/4(d/dt_phase)
  Constant17/1 -> delay_gen0/8(din1)
  Slice18/1 -> Concat4/1
  Slice17/1 -> Concat4/2
  Concat4/1 -> delay_gen0/5(delay)
  Slice15/1 -> delay_gen0/6(d/dt_delay)
  Constant19/1 -> delay_gen0/9(invert_slope)
  [cd_en1] -> delay_gen1/2(en)
  Slice21/1 -> delay_gen1/3(phase)
  Slice24/1 -> delay_gen1/4(d/dt_phase)
  Constant21/1 -> delay_gen1/8(din1)
  Slice23/1 -> Concat5/1
  Slice22/1 -> Concat5/2
  Concat5/1 -> delay_gen1/5(delay)
  Slice20/1 -> delay_gen1/6(d/dt_delay)
  Constant22/1 -> delay_gen1/9(invert_slope)
  fft_wideband_real1/4(of) -> [fft_or1]
  [adc0] -> decat2/1(i1)
  decat2/1(o1) -> auto_shutoff0/1(In1)
  decat2/2(o2) -> auto_shutoff0/2(In2)
  decat2/3(o3) -> auto_shutoff0/3(In3)
  decat2/4(o4) -> auto_shutoff0/4(In4)
  [clr_status] -> auto_shutoff0/5(rst)
  auto_shutoff0/1(en) -> [adc_bad0]
  katadc0/11(sync0) -> Concat8/1
  katadc0/12(sync1) -> Concat8/2
  katadc0/13(sync2) -> Concat8/3
  katadc0/14(sync3) -> Concat8/4
  Concat8/1 -> [sync_raw0]
  Slice35/1 -> Logical/1
  Slice36/1 -> Logical/2
  Slice40/1 -> Logical/3
  Slice45/1 -> Logical/4
  [sync_raw0] -> Slice35/1, Slice45/1, Slice40/1, Slice36/1
  [sync_val0] -> Subsystem7/8(sync_val)
  [adc1] -> decat3/1(i1)
  decat3/1(o1) -> auto_shutoff1/1(In1)
  decat3/2(o2) -> auto_shutoff1/2(In2)
  decat3/3(o3) -> auto_shutoff1/3(In3)
  decat3/4(o4) -> auto_shutoff1/4(In4)
  [clr_status] -> auto_shutoff1/5(rst)
  auto_shutoff1/1(en) -> [adc_bad1]
  arm11/1 -> [adc_protect_disable]
  [adc_bad_latch0] -> Inverter1/1
  Inverter1/1 -> Logical6/1
  [adc_protect_disable] -> Logical6/2
  Logical8/1 -> [adc_en0], katadc0/5(en0)
  Logical6/1 -> Logical8/1
  Slice29/1 -> Logical8/2
  Slice30/1 -> katadc0/6(atten0)
  [adc_bad_latch1] -> Inverter2/1
  Inverter2/1 -> Logical9/1
  [adc_protect_disable] -> Logical9/2
  Logical9/1 -> Logical10/1
  Slice33/1 -> Logical10/2
  Logical10/1 -> [adc_en1], katadc0/7(en1)
  Slice34/1 -> katadc0/8(atten1)
  [mrst] -> edge_detect/1(in)
  edge_detect/1(out) -> Delay/1
  [mrst] -> cd_tr0/1(rst)
  Logical11/1 -> cd_tr0/3(arm)
  [cd_local_time] -> cd_tr0/4(current_time)
  [mrst] -> fd_tr0/1(rst)
  Logical12/1 -> fd_tr0/3(arm)
  [fd_local_time] -> fd_tr0/4(current_time)
  Slice38/1 -> AddSub/1
  [sync_val0] -> AddSub/2
  AddSub/1 -> Concat22/3
  Constant25/1 -> trig_level/1
  trig_level/1 -> trig0/3(trig_pnt), trig1/3(trig_pnt)
  [data_adc1] -> trig1/2(adc_data)
  [sync_raw0] -> Register3/1
  [adc_sync0] -> Logical5/1
  Logical5/1 -> Register3/2
  [mrst] -> Logical5/2
  Register3/1 -> convert/1(in)
  convert/1(Out1) -> [sync_val0]
  gbe_tx_cnt0/1(sim_reg_out) -> Terminator3/1
  Delay14/1(q) -> gbe_tx_cnt0/1(reg_out)
  trig1/3(trig) -> [trig_adc1]
  Delay8/1 -> adc_sum_sq0/1(reg_out)
  Delay12/1 -> adc_sum_sq1/1(reg_out)
  trig1/2(data) -> [trig_data1]
  [trig_data0] -> adc_snap0/1(din)
  trig0/2(data) -> [trig_data0]
  trig0/3(trig) -> [trig_adc0]
  [sync] -> trig1/1(synci)
  [data_adc0] -> trig0/2(adc_data)
  trig1/1(synco) -> Terminator5/1
  [pps] -> Counter1/1, Counter3/2, Register19/2
  Delay7/1 -> Slice1/1, Slice/1
  Delay/1 -> [load_now]
  Slice7/1 -> [arm0]
  [load_now] -> cd_tr0/2(load_now), Logical11/1
  [arm0] -> Logical11/2
  [arm0] -> Logical12/2
  [load_now] -> Logical12/1, fd_tr0/2(load_now)
  cd_tr0/2(ld_count) -> Terminator15/1
  cd_tr0/3(value) -> [cd_val0]
  cd_tr0/4(enable) -> [cd_en0]
  Concat9/1 -> [ld_time0]
  [ld_time0] -> cd_tr0/5(load_time)
  Concat22/1 -> [ld_val0]
  fd_tr0/1(arm_count) -> Convert4/1
  fd_tr0/2(ld_count) -> Convert5/1
  [ld_val0] -> cd_tr0/6(load_value)
  [ld_time0] -> fd_tr0/5(load_time)
  [ld_val0] -> fd_tr0/6(load_value)
  a1_fd0/1 -> Slice4/1, Slice5/1
  cd_tr1/1(arm_count) -> Terminator16/1
  [mrst] -> cd_tr1/1(rst)
  Logical19/1 -> cd_tr1/3(arm)
  [cd_local_time] -> cd_tr1/4(current_time)
  [load_now] -> Logical19/1, cd_tr1/2(load_now)
  [arm1] -> Logical19/2
  cd_tr1/2(ld_count) -> Terminator18/1
  cd_tr1/3(value) -> [cd_val1]
  cd_tr1/4(enable) -> [cd_en1]
  [ld_time1] -> cd_tr1/5(load_time)
  [ld_val1] -> cd_tr1/6(load_value)
  fd_fs_tvg0/4(dout1) -> bus_create/3(in3), Subsystem4/3(din1)
  bus_create/1(bus_out) -> fd_tr0/7(din)
  fd_tr0/5(dout) -> bus_expand1/1(bus_in)
  bus_expand1/2(out2) -> Delay15/1
  bus_expand1/3(lsb_out1) -> Delay16/1
  eq0/1(data_out) -> bus_expand2/1(bus_in)
  Delay13/1 -> quant0/5(sync_in)
  Delay15/1 -> quant0/6(din0)
  Delay16/1 -> quant0/7(din1)
  bus_expand2/1(msb_out4) -> quant0/1(real_in0)
  bus_expand2/2(out3) -> quant0/2(imag_in0)
  bus_expand2/3(out2) -> quant0/3(real_in1)
  bus_expand2/4(lsb_out1) -> quant0/4(real_in2)
  [mrst] -> fd_tr1/1(rst)
  Logical13/1 -> fd_tr1/3(arm)
  [fd_local_time] -> fd_tr1/4(current_time)
  [arm1] -> Logical13/2
  [load_now] -> fd_tr1/2(load_now), Logical13/1
  fd_tr1/1(arm_count) -> Convert6/1
  fd_tr1/2(ld_count) -> Convert7/1
  [ld_time1] -> fd_tr1/5(load_time)
  [ld_val1] -> fd_tr1/6(load_value)
  fd_fs_tvg1/1(sync_out) -> bus_create1/1(in1)
  fd_fs_tvg1/2(dout0) -> bus_create1/2(in2)
  fd_fs_tvg1/3(dout1) -> bus_create1/3(in3)
  bus_create1/1(bus_out) -> fd_tr1/7(din)
  fd_tr1/5(dout) -> bus_expand3/1(bus_in)
  bus_expand3/3(lsb_out1) -> Delay19/1
  quant1/2(dout0) -> Concat3/1
  quant1/3(dout1) -> Concat3/2
  quant1/1(sync_out) -> [quant1_sync]
  quant1/4(of) -> [quant_or1]
  Concat3/1 -> [quant1_data]
  bus_expand3/1(msb_out3) -> Delay17/1, Counter2/1
  Counter2/1 -> eq1/1(addr)
  Constant10/1 -> eq1/2(data_in)
  Constant11/1 -> eq1/3(we)
  bus_expand3/2(out2) -> Delay18/1
  eq1/1(data_out) -> bus_expand4/1(bus_in)
  Delay17/1 -> quant1/5(sync_in)
  Delay18/1 -> quant1/6(din0)
  Delay19/1 -> quant1/7(din1)
  bus_expand4/1(msb_out4) -> quant1/1(real_in0)
  bus_expand4/2(out3) -> quant1/2(imag_in0)
  bus_expand4/3(out2) -> quant1/3(real_in1)
  bus_expand4/4(lsb_out1) -> quant1/4(real_in2)
  cd_tr1/5(dout) -> delay_gen1/7(din0)
  [data_adc1] -> cd_tr1/7(din)
  [mrst] -> gpio_tr/1(rst)
  Logical15/1 -> gpio_tr/3(arm)
  [cd_local_time] -> gpio_tr/4(current_time)
  [load_now] -> gpio_tr/2(load_now), Logical15/1
  [arm0] -> Logical15/2
  [ld_time0] -> gpio_tr/5(load_time)
  Constant34/1 -> gpio_tr/6(load_value)
  [timing_pps] -> gpio_tr/7(din)
  gpio_tr/5(dout) -> Delay28/1
  gpio_tr/1(arm_count) -> Terminator19/1
  gpio_tr/2(ld_count) -> Terminator21/1
  Constant24/1 -> adc_snap0/2(we)
  [trig_sync] -> adc_snap0/3(trig)
  [trig_adc0] -> adc_snap0/4(stop)
  [timing_pps] -> Concat6/1
  [cd_local_time] -> Slice14/1
  Concat6/1 -> trig0/1(synci)
  trig0/1(synco) -> bus_expand/1(bus_in)
  bus_expand/1(msb_out2) -> [trig_sync]
  Slice14/1 -> Concat6/2
  bus_expand/2(lsb_out1) -> [timestamp]
  [timestamp] -> adc_snap0/5(vin)
  [trig_data1] -> adc_snap1/1(din)
  [trig_adc1] -> adc_snap1/4(stop)
  [timestamp] -> adc_snap1/5(vin)
  [trig_sync] -> scopes/1(sync)
  [timestamp] -> scopes/3(time)
  [trig_data0] -> scopes/2(data)
  [adc_en0] -> Inverter5/1
  [adc_en1] -> Inverter6/1
  fd_fs_tvg0/3(dout0) -> bus_create/2(in2), Subsystem4/2(din0)
  fd_fs_tvg0/2(sync_out) -> bus_create/1(in1), Subsystem4/1(sync)
  fd_fs_tvg0/1(time_o) -> [fd_local_time]
  [fd_local_time] -> Subsystem4/4(time)
  [mrst] -> tvg_tr/1(rst)
  Logical20/1 -> tvg_tr/3(arm)
  [arm0] -> Logical20/2
  [load_now] -> tvg_tr/2(load_now), Logical20/1
  [ld_time0] -> tvg_tr/5(load_time)
  Constant35/1 -> tvg_tr/6(load_value)
  Constant14/1 -> tvg_tr/7(din)
  tvg_tr/5(dout) -> Terminator23/1
  tvg_tr/1(arm_count) -> Terminator26/1
  tvg_tr/2(ld_count) -> Terminator27/1
  tvg_tr/3(value) -> Terminator29/1
  tvg_tr/4(enable) -> [tvg_tr_en]
  [fd_fs_tvg] -> Register2/1
  Delay20/1 -> fd_fs_tvg0/2(sync)
  Delay21/1 -> fd_fs_tvg0/5(din1)
  Delay22/1 -> fd_fs_tvg0/4(din0)
  Delay24/1 -> fd_fs_tvg0/1(time)
  Delay25/1 -> fd_fs_tvg1/2(sync)
  Delay26/1 -> fd_fs_tvg1/3(din0)
  Delay27/1 -> fd_fs_tvg1/4(din1)
  Logical7/1 -> leds/1(warning)
  [sync] -> leds/4(sync_led)
  Logical4/1 -> leds/6(comms)
  [pps] -> leds/5(pps)
  [mrst] -> leds/3(rst)
  [fancy_en] -> leds/2(fancy_en)
  [xaui_ldn0] -> Logical4/1
  [xaui_of0] -> Logical4/2
  [adc_en0] -> Inverter3/1
  [adc_en1] -> Inverter4/1
  [adc_or1] -> Logical16/1
  [fft_or1] -> Logical16/2
  [adc_or0] -> Logical17/1
  [fft_or0] -> Logical17/2
  Logical17/1 -> leds/9(or0)
  Logical16/1 -> leds/10(or1)
  [adc_en0] -> leds/7(adc_en0)
  [adc_en1] -> leds/8(adc_en1)
  [xaui_of0] -> Logical7/2
  [xaui_ldn0] -> Logical7/1
  [adc_sync0] -> adc_scope/1(In1)
  [adc0] -> adc_scope/2(In2)
  [adc1] -> adc_scope/3(In3)
  [sync] -> Concat10/1
  [data_adc0] -> Concat10/2
  Concat10/1 -> cd_tr0/7(din)
  cd_tr0/5(dout) -> bus_expand5/1(bus_in)
  bus_expand5/1(msb_out2) -> delay_gen0/1(sync_in), delay_gen1/1(sync_in)
  bus_expand5/2(lsb_out1) -> delay_gen0/7(din0)
  gpio_tr/3(value) -> Terminator28/1
  gpio_tr/4(enable) -> Register4/2
  [tvg_en] -> Register2/2
  [tvg_tr_en] -> fd_fs_tvg0/6(val_en)
  Constant36/1 -> Relational/2
  Constant37/1 -> Relational1/2
  Relational/1 -> Logical21/1
  Relational1/1 -> Logical21/2
  Logical21/1 -> [clk_bad]
  [clk_bad] -> Subsystem7/10(clk_bad)
  Inverter5/1 -> Subsystem7/9(adc_disable)
  [clr_status] -> Subsystem1/1(clr)
  [xaui_ldn0] -> Subsystem1/2(xuai_ldn)
  [xaui_of0] -> Subsystem1/3(xaui_of)
  [ct_err0] -> Subsystem1/4(ct_err)
  [adc_or1] -> Subsystem1/5(adc_or)
  [fft_or1] -> Subsystem1/6(fft_or)
  [quant_or1] -> Subsystem1/7(quant_or)
  [sync_val0] -> Subsystem1/8(sync_val)
  Inverter6/1 -> Subsystem1/9(adc_disable)
  [clk_bad] -> Subsystem1/10(clk_bad)
  Subsystem3/1(data_out) -> snap_gbe_tx0/1(din)
  Subsystem3/3(trig_out) -> snap_gbe_tx0/3(trig)
  Subsystem3/2(we_out) -> snap_gbe_tx0/2(we)
  [trig_sync] -> adc_snap1/3(trig)
  Constant1/1 -> adc_snap1/2(we)
  [arm0] -> edge_detect2/1(in)
  Constant38/1 -> Register4/1
  Register4/1 -> Subsystem5/1(In1)
  edge_detect2/1(out) -> Register4/3
  [adc0] -> Concat/2
  [adc1] -> Concat/3
  [adc_sync0] -> Concat/1
  timing/3(data_out) -> bus_expand6/1(bus_in)
  bus_expand6/3(lsb_out1) -> [data_adc1]
  bus_expand6/2(out2) -> [data_adc0]
  bus_expand6/1(msb_out3) -> [timing_pps]
  Delay28/1 -> Subsystem5/2(din)
  Inverter3/1 -> Logical7/3
  Inverter4/1 -> Logical7/4
  [clk_bad] -> Logical7/5
  delay_tr_status0/1(sim_reg_out) -> Terminator17/1
  Convert4/1 -> Concat13/1
  Concat13/1 -> delay_tr_status0/1(reg_out)
  Convert5/1 -> Concat13/2
  delay_tr_status1/1(sim_reg_out) -> Terminator6/1
  Convert6/1 -> Concat14/1
  Concat14/1 -> delay_tr_status1/1(reg_out)
  Convert7/1 -> Concat14/2
  Constant23/1 -> [dram_not_ready]
  [dram_not_ready] -> Subsystem1/11(dram_bad)
  [dram_not_ready] -> Subsystem7/11(dram_bad)
  [ct_err0] -> Logical7/7
  [dram_not_ready] -> Logical7/6
  ct/3(data_out) -> pkt_cont_tvg0/4(din)
  [board_id] -> pkt_cont_tvg0/5(antenna)
  Register9/1 -> [adc_bad_latch0]
  [adc_bad0] -> Register9/1, Register9/3
  [clr_adc_bad] -> Register9/2
  Register5/1 -> [adc_bad_latch1]
  [adc_bad1] -> Register5/3, Register5/1
  [clr_adc_bad] -> Register5/2
  Subsystem7/1(status) -> fstatus0/1(reg_out)
  arm12/1 -> posedge3/1
  posedge3/1 -> [clr_adc_bad]
  Constant13/1 -> ld_time_msw1/1
  Constant6/1 -> ld_time_lsw1/1
  ld_time_msw1/1 -> Slice32/1, Slice37/1
  Slice37/1 -> Concat2/1
  ld_time_lsw1/1 -> Concat2/2
  Constant12/1 -> coarse_delay1/1
  Constant16/1 -> a0_fd1/1
  Constant15/1 -> a1_fd1/1
  a0_fd1/1 -> Slice13/1, Slice25/1
  Slice28/1 -> Concat1/4
  Slice31/1 -> Concat1/5
  coarse_delay1/1 -> Slice27/1
  Slice13/1 -> Concat1/1
  Slice25/1 -> Concat1/2
  Slice27/1 -> AddSub1/1
  [sync_val0] -> AddSub1/2
  AddSub1/1 -> Concat1/3
  Slice32/1 -> [arm1]
  Concat2/1 -> [ld_time1]
  Concat1/1 -> [ld_val1]
  a1_fd1/1 -> Slice31/1, Slice28/1
  Subsystem1/1(status) -> fstatus1/1(reg_out)
  delay_wideband_prog1/3(data_out2) -> pfb_fir_real/7(pol2_in2)
  delay_wideband_prog1/4(data_out3) -> pfb_fir_real/8(pol2_in3)
  delay_wideband_prog1/5(data_out4) -> pfb_fir_real/9(pol2_in4)
  delay_wideband_prog1/2(data_out1) -> pfb_fir_real/6(pol2_in1)
  pfb_fir_real/8(pol2_out3) -> a0p1_1st_shift/4(din3)
  pfb_fir_real/6(pol2_out1) -> a0p1_1st_shift/2(din1)
  pfb_fir_real/7(pol2_out2) -> a0p1_1st_shift/3(din2)
  pfb_fir_real/9(pol2_out4) -> a0p1_1st_shift/5(din4)
